simulink model "NeuroControlExamen"  (R2023b)
settings: Solver=VariableStepAuto  StartTime=0.0  StopTime=10.0  RelTol=1e-3
(part 2 of 3)

== matlab function NeuroControlExamen/Dinamica4 ==
  data: q input; qdd output; qd input; tau input
function qdd = fcn(q, qd, tau)

q1=q(1);
q2=q(2);
q3=q(3);
q1_d=qd(1);
q2_d=qd(2);
q3_d=qd(3);

m1 = 1;
m2 = 1;
m3 = 1;
l1 = 1;
l2 = 1;
l3 = 1;
lc1 = 0.5;
lc2 = 0.5;
lc3 = 0.5;
Ixx1 = 0.02;
Ixx2 = 0.02;
Ixx3 = 0.02;
Iyy1 = 0.02;
Iyy2 = 0.02;
Iyy3 = 0.02;
Izz1 = 0.02;
Izz2 = 0.02;
Izz3 = 0.02;

g = 9.81;

H = [Iyy1 + Ixx3*(cos(q2)*sin(q3) + cos(q3)*sin(q2))^2 + Iyy3*(cos(q2)*cos(q3) - sin(q2)*sin(q3))^2 + Iyy2*cos(q2)^2 + 2*m3*(l2*cos(q2)*sin(q1) + lc3*cos(q2)*cos(q3)*sin(q1) - lc3*sin(q1)*sin(q2)*sin(q3))^2 + Ixx2*sin(q2)^2 + lc2^2*m2*cos(q1)^2*cos(q2)^2 + lc2^2*m2*cos(q2)^2*sin(q1)^2, sin(q1)*(Ixx2*cos(q1)*cos(q2)*sin(q2) - Iyy2*cos(q1)*cos(q2)*sin(q2)) - cos(q1)*(Ixx2*cos(q2)*sin(q1)*sin(q2) - Iyy2*cos(q2)*sin(q1)*sin(q2)) + sin(q1)*(Ixx3*(cos(q1)*cos(q2)*cos(q3) - cos(q1)*sin(q2)*sin(q3))*(cos(q2)*sin(q3) + cos(q3)*sin(q2)) - Iyy3*(cos(q1)*cos(q2)*sin(q3) + cos(q1)*cos(q3)*sin(q2))*(cos(q2)*cos(q3) - sin(q2)*sin(q3))) + cos(q1)*(Ixx3*(sin(q1)*sin(q2)*sin(q3) - cos(q2)*cos(q3)*sin(q1))*(cos(q2)*sin(q3) + cos(q3)*sin(q2)) + Iyy3*(cos(q2)*sin(q1)*sin(q3) + cos(q3)*sin(q1)*sin(q2))*(cos(q2)*cos(q3) - sin(q2)*sin(q3))) + 2*m3*(l2*cos(q1)*sin(q2) + lc3*cos(q1)*cos(q2)*sin(q3) + lc3*cos(q1)*cos(q3)*sin(q2))*(l2*cos(q2)*sin(q1) + lc3*cos(q2)*cos(q3)*sin(q1) - lc3*sin(q1)*sin(q2)*sin(q3)), sin(q1)*(Ixx3*(cos(q1)*cos(q2)*cos(q3) - cos(q1)*sin(q2)*sin(q3))*(cos(q2)*sin(q3) + cos(q3)*sin(q2)) - Iyy3*(cos(q1)*cos(q2)*sin(q3) + cos(q1)*cos(q3)*sin(q2))*(cos(q2)*cos(q3) - sin(q2)*sin(q3))) + cos(q1)*(Ixx3*(sin(q1)*sin(q2)*sin(q3) - cos(q2)*cos(q3)*sin(q1))*(cos(q2)*sin(q3) + cos(q3)*sin(q2)) + Iyy3*(cos(q2)*sin(q1)*sin(q3) + cos(q3)*sin(q1)*sin(q2))*(cos(q2)*cos(q3) - sin(q2)*sin(q3))) + 2*m3*(lc3*cos(q1)*cos(q2)*sin(q3) + lc3*cos(q1)*cos(q3)*sin(q2))*(l2*cos(q2)*sin(q1) + lc3*cos(q2)*cos(q3)*sin(q1) - lc3*sin(q1)*sin(q2)*sin(q3));
     sin(q1)*(Ixx2*cos(q1)*cos(q2)*sin(q2) - Iyy2*cos(q1)*cos(q2)*sin(q2)) - cos(q1)*(Ixx2*cos(q2)*sin(q1)*sin(q2) - Iyy2*cos(q2)*sin(q1)*sin(q2)) + sin(q1)*(Ixx3*(cos(q1)*cos(q2)*cos(q3) - cos(q1)*sin(q2)*sin(q3))*(cos(q2)*sin(q3) + cos(q3)*sin(q2)) - Iyy3*(cos(q1)*cos(q2)*sin(q3) + cos(q1)*cos(q3)*sin(q2))*(cos(q2)*cos(q3) - sin(q2)*sin(q3))) + cos(q1)*(Ixx3*(sin(q1)*sin(q2)*sin(q3) - cos(q2)*cos(q3)*sin(q1))*(cos(q2)*sin(q3) + cos(q3)*sin(q2)) + Iyy3*(cos(q2)*sin(q1)*sin(q3) + cos(q3)*sin(q1)*sin(q2))*(cos(q2)*cos(q3) - sin(q2)*sin(q3))) + 2*m3*(l2*cos(q1)*sin(q2) + lc3*cos(q1)*cos(q2)*sin(q3) + lc3*cos(q1)*cos(q3)*sin(q2))*(l2*cos(q2)*sin(q1) + lc3*cos(q2)*cos(q3)*sin(q1) - lc3*sin(q1)*sin(q2)*sin(q3)), sin(q1)*(sin(q1)*(Ixx3*(cos(q1)*cos(q2)*cos(q3) - cos(q1)*sin(q2)*sin(q3))^2 + Iyy3*(cos(q1)*cos(q2)*sin(q3) + cos(q1)*cos(q3)*sin(q2))^2 + Izz3*sin(q1)^2) + cos(q1)*(Ixx3*(cos(q1)*cos(q2)*cos(q3) - cos(q1)*sin(q2)*sin(q3))*(sin(q1)*sin(q2)*sin(q3) - cos(q2)*cos(q3)*sin(q1)) - Iyy3*(cos(q1)*cos(q2)*sin(q3) + cos(q1)*cos(q3)*sin(q2))*(cos(q2)*sin(q1)*sin(q3) + cos(q3)*sin(q1)*sin(q2)) + Izz3*cos(q1)*sin(q1))) + cos(q1)*(cos(q1)*(Ixx3*(sin(q1)*sin(q2)*sin(q3) - cos(q2)*cos(q3)*sin(q1))^2 + Iyy3*(cos(q2)*sin(q1)*sin(q3) + cos(q3)*sin(q1)*sin(q2))^2 + Izz3*cos(q1)^2) + sin(q1)*(Ixx3*(cos(q1)*cos(q2)*cos(q3) - cos(q1)*sin(q2)*sin(q3))*(sin(q1)*sin(q2)*sin(q3) - cos(q2)*cos(q3)*sin(q1)) - Iyy3*(cos(q1)*cos(q2)*sin(q3) + cos(q1)*cos(q3)*sin(q2))*(cos(q2)*sin(q1)*sin(q3) + cos(q3)*sin(q1)*sin(q2)) + Izz3*cos(q1)*sin(q1))) - cos(q1)*(sin(q1)*(Ixx2*cos(q1)*cos(q2)^2*sin(q1) - Izz2*cos(q1)*sin(q1) + Iyy2*cos(q1)*sin(q1)*sin(q2)^2) - cos(q1)*(Izz2*cos(q1)^2 + Ixx2*cos(q2)^2*sin(q1)^2 + Iyy2*sin(q1)^2*sin(q2)^2)) - sin(q1)*(cos(q1)*(Ixx2*cos(q1)*cos(q2)^2*sin(q1) - Izz2*cos(q1)*sin(q1) + Iyy2*cos(q1)*sin(q1)*sin(q2)^2) - sin(q1)*(Ixx2*cos(q1)^2*cos(q2)^2 + Iyy2*cos(q1)^2*sin(q2)^2 + Izz2*sin(q1)^2)) + 2*m3*(l2*cos(q1)*sin(q2) + lc3*cos(q1)*cos(q2)*sin(q3) + lc3*cos(q1)*cos(q3)*sin(q2))^2 + m3*(cos(q2)*(l1 + l2) + lc3*cos(q2)*cos(q3) - lc3*sin(q2)*sin(q3))^2 + m2*cos(q2)^2*(l1 + lc2)^2 + lc2^2*m2*cos(q1)^2*sin(q2)^2 + lc2^2*m2*sin(q1)^2*sin(q2)^2, sin(q1)*(sin(q1)*(Ixx3*(cos(q1)*cos(q2)*cos(q3) - cos(q1)*sin(q2)*sin(q3))^2 + Iyy3*(cos(q1)*cos(q2)*sin(q3) + cos(q1)*cos(q3)*sin(q2))^2 + Izz3*sin(q1)^2) + cos(q1)*(Ixx3*(cos(q1)*cos(q2)*cos(q3) - cos(q1)*sin(q2)*sin(q3))*(sin(q1)*sin(q2)*sin(q3) - cos(q2)*cos(q3)*sin(q1)) - Iyy3*(cos(q1)*cos(q2)*sin(q3) + cos(q1)*cos(q3)*sin(q2))*(cos(q2)*sin(q1)*sin(q3) + cos(q3)*sin(q1)*sin(q2)) + Izz3*cos(q1)*sin(q1))) + cos(q1)*(cos(q1)*(Ixx3*(sin(q1)*sin(q2)*sin(q3) - cos(q2)*cos(q3)*sin(q1))^2 + Iyy3*(cos(q2)*sin(q1)*sin(q3) + cos(q3)*sin(q1)*sin(q2))^2 + Izz3*cos(q1)^2) + sin(q1)*(Ixx3*(cos(q1)*cos(q2)*cos(q3) - cos(q1)*sin(q2)*sin(q3))*(sin(q1)*sin(q2)*sin(q3) - cos(q2)*cos(q3)*sin(q1)) - Iyy3*(cos(q1)*cos(q2)*sin(q3) + cos(q1)*cos(q3)*sin(q2))*(cos(q2)*sin(q1)*sin(q3) + cos(q3)*sin(q1)*sin(q2)) + Izz3*cos(q1)*sin(q1))) + m3*(lc3*cos(q2)*cos(q3) - lc3*sin(q2)*sin(q3))*(cos(q2)*(l1 + l2) + lc3*cos(q2)*cos(q3) - lc3*sin(q2)*sin(q3)) + 2*m3*(lc3*cos(q1)*cos(q2)*sin(q3) + lc3*cos(q1)*cos(q3)*sin(q2))*(l2*cos(q1)*sin(q2) + lc3*cos(q1)*cos(q2)*sin(q3) + lc3*cos(q1)*cos(q3)*sin(q2));
     sin(q1)*(Ixx3*(cos(q1)*cos(q2)*cos(q3) - cos(q1)*sin(q2)*sin(q3))*(cos(q2)*sin(q3) + cos(q3)*sin(q2)) - Iyy3*(cos(q1)*cos(q2)*sin(q3) + cos(q1)*cos(q3)*sin(q2))*(cos(q2)*cos(q3) - sin(q2)*sin(q3))) + cos(q1)*(Ixx3*(sin(q1)*sin(q2)*sin(q3) - cos(q2)*cos(q3)*sin(q1))*(cos(q2)*sin(q3) + cos(q3)*sin(q2)) + Iyy3*(cos(q2)*sin(q1)*sin(q3) + cos(q3)*sin(q1)*sin(q2))*(cos(q2)*cos(q3) - sin(q2)*sin(q3))) + 2*m3*(lc3*cos(q1)*cos(q2)*sin(q3) + lc3*cos(q1)*cos(q3)*sin(q2))*(l2*cos(q2)*sin(q1) + lc3*cos(q2)*cos(q3)*sin(q1) - lc3*sin(q1)*sin(q2)*sin(q3)), sin(q1)*(sin(q1)*(Ixx3*(cos(q1)*cos(q2)*cos(q3) - cos(q1)*sin(q2)*sin(q3))^2 + Iyy3*(cos(q1)*cos(q2)*sin(q3) + cos(q1)*cos(q3)*sin(q2))^2 + Izz3*sin(q1)^2) + cos(q1)*(Ixx3*(cos(q1)*cos(q2)*cos(q3) - cos(q1)*sin(q2)*sin(q3))*(sin(q1)*sin(q2)*sin(q3) - cos(q2)*cos(q3)*sin(q1)) - Iyy3*(cos(q1)*cos(q2)*sin(q3) + cos(q1)*cos(q3)*sin(q2))*(cos(q2)*sin(q1)*sin(q3) + cos(q3)*sin(q1)*sin(q2)) + Izz3*cos(q1)*sin(q1))) + cos(q1)*(cos(q1)*(Ixx3*(sin(q1)*sin(q2)*sin(q3) - cos(q2)*cos(q3)*sin(q1))^2 + Iyy3*(cos(q2)*sin(q1)*sin(q3) + cos(q3)*sin(q1)*sin(q2))^2 + Izz3*cos(q1)^2) + sin(q1)*(Ixx3*(cos(q1)*cos(q2)*cos(q3) - cos(q1)*sin(q2)*sin(q3))*(sin(q1)*sin(q2)*sin(q3) - cos(q2)*cos(q3)*sin(q1)) - Iyy3*(cos(q1)*cos(q2)*sin(q3) + cos(q1)*cos(q3)*sin(q2))*(cos(q2)*sin(q1)*sin(q3) + cos(q3)*sin(q1)*sin(q2)) + Izz3*cos(q1)*sin(q1))) + m3*(lc3*cos(q2)*cos(q3) - lc3*sin(q2)*sin(q3))*(cos(q2)*(l1 + l2) + lc3*cos(q2)*cos(q3) - lc3*sin(q2)*sin(q3)) + 2*m3*(lc3*cos(q1)*cos(q2)*sin(q3) + lc3*cos(q1)*cos(q3)*sin(q2))*(l2*cos(q1)*sin(q2) + lc3*cos(q1)*cos(q2)*sin(q3) + lc3*cos(q1)*cos(q3)*sin(q2)), sin(q1)*(sin(q1)*(Ixx3*(cos(q1)*cos(q2)*cos(q3) - cos(q1)*sin(q2)*sin(q3))^2 + Iyy3*(cos(q1)*cos(q2)*sin(q3) + cos(q1)*cos(q3)*sin(q2))^2 + Izz3*sin(q1)^2) + cos(q1)*(Ixx3*(cos(q1)*cos(q2)*cos(q3) - cos(q1)*sin(q2)*sin(q3))*(sin(q1)*sin(q2)*sin(q3) - cos(q2)*cos(q3)*sin(q1)) - Iyy3*(cos(q1)*cos(q2)*sin(q3) + cos(q1)*cos(q3)*sin(q2))*(cos(q2)*sin(q1)*sin(q3) + cos(q3)*sin(q1)*sin(q2)) + Izz3*cos(q1)*sin(q1))) + 2*m3*(lc3*cos(q1)*cos(q2)*sin(q3) + lc3*cos(q1)*cos(q3)*sin(q2))^2 + cos(q1)*(cos(q1)*(Ixx3*(sin(q1)*sin(q2)*sin(q3) - cos(q2)*cos(q3)*sin(q1))^2 + Iyy3*(cos(q2)*sin(q1)*sin(q3) + cos(q3)*sin(q1)*sin(q2))^2 + Izz3*cos(q1)^2) + sin(q1)*(Ixx3*(cos(q1)*cos(q2)*cos(q3) - cos(q1)*sin(q2)*sin(q3))*(sin(q1)*sin(q2)*sin(q3) - cos(q2)*cos(q3)*sin(q1)) - Iyy3*(cos(q1)*cos(q2)*sin(q3) + cos(q1)*cos(q3)*sin(q2))*(cos(q2)*sin(q1)*sin(q3) + cos(q3)*sin(q1)*sin(q2)) + Izz3*cos(q1)*sin(q1))) + m3*(lc3*cos(q2)*cos(q3) - lc3*sin(q2)*sin(q3))^2];
 
g_q = [g*m2*(lc2*cos(q1 + q2) + l1*cos(q1)) + g*lc1*m1*cos(q1);
       g*lc2*m2*cos(q1 + q2);
       0];

C = [2*m3*q1_d*(l2*cos(q1)*cos(q2) + lc3*cos(q1)*cos(q2)*cos(q3) - lc3*cos(q1)*sin(q2)*sin(q3))*(l2*cos(q2)*sin(q1) + lc3*cos(q2)*cos(q3)*sin(q1) - lc3*sin(q1)*sin(q2)*sin(q3)) - q2_d*(2*m3*(l2*cos(q2)*sin(q1) + lc3*cos(q2)*cos(q3)*sin(q1) - lc3*sin(q1)*sin(q2)*sin(q3))*(l2*sin(q1)*sin(q2) + lc3*cos(q2)*sin(q1)*sin(q3) + lc3*cos(q3)*sin(q1)*sin(q2)) - Ixx2*cos(q2)*sin(q2) + Iyy2*cos(q2)*sin(q2) - Ixx3*(cos(q2)*sin(q3) + cos(q3)*sin(q2))*(cos(q2)*cos(q3) - sin(q2)*sin(q3)) + Iyy3*(cos(q2)*sin(q3) + cos(q3)*sin(q2))*(cos(q2)*cos(q3) - sin(q2)*sin(q3)) + lc2^2*m2*cos(q1)^2*cos(q2)*sin(q2) + lc2^2*m2*cos(q2)*sin(q1)^2*sin(q2)) - q3_d*(2*m3*(lc3*cos(q2)*sin(q1)*sin(q3) + lc3*cos(q3)*sin(q1)*sin(q2))*(l2*cos(q2)*sin(q1) + lc3*cos(q2)*cos(q3)*sin(q1) - lc3*sin(q1)*sin(q2)*sin(q3)) - Ixx3*(cos(q2)*sin(q3) + cos(q3)*sin(q2))*(cos(q2)*cos(q3) - sin(q2)*sin(q3)) + Iyy3*(cos(q2)*sin(q3) + cos(q3)*sin(q2))*(cos(q2)*cos(q3) - sin(q2)*sin(q3))), q2_d*((sin(q1)*(cos(q1)*(Ixx3*(sin(q1)*sin(q2)*sin(q3) - cos(q2)*cos(q3)*sin(q1))^2 + Iyy3*(cos(q2)*sin(q1)*sin(q3) + cos(q3)*sin(q1)*sin(q2))^2 + Izz3*cos(q1)^2) + sin(q1)*(Ixx3*(cos(q1)*cos(q2)*cos(q3) - cos(q1)*sin(q2)*sin(q3))*(sin(q1)*sin(q2)*sin(q3) - cos(q2)*cos(q3)*sin(q1)) - Iyy3*(cos(q1)*cos(q2)*sin(q3) + cos(q1)*cos(q3)*sin(q2))*(cos(q2)*sin(q1)*sin(q3) + cos(q3)*sin(q1)*sin(q2)) + Izz3*cos(q1)*sin(q1))))/2 - (sin(q1)*(cos(q1)*(Ixx3*(cos(q1)*cos(q2)*cos(q3) - cos(q1)*sin(q2)*sin(q3))^2 + Iyy3*(cos(q1)*cos(q2)*sin(q3) + cos(q1)*cos(q3)*sin(q2))^2 + Izz3*sin(q1)^2) - sin(q1)*(Ixx3*(cos(q1)*cos(q2)*cos(q3) - cos(q1)*sin(q2)*sin(q3))*(sin(q1)*sin(q2)*sin(q3) - cos(q2)*cos(q3)*sin(q1)) - Iyy3*(cos(q1)*cos(q2)*sin(q3) + cos(q1)*cos(q3)*sin(q2))*(cos(q2)*sin(q1)*sin(q3) + cos(q3)*sin(q1)*sin(q2)) + Izz3*cos(q1)*sin(q1)) + sin(q1)*(2*Ixx3*(cos(q1)*cos(q2)*cos(q3) - cos(q1)*sin(q2)*sin(q3))*(sin(q1)*sin(q2)*sin(q3) - cos(q2)*cos(q3)*sin(q1)) - 2*Iyy3*(cos(q1)*cos(q2)*sin(q3) + cos(q1)*cos(q3)*sin(q2))*(cos(q2)*sin(q1)*sin(q3) + cos(q3)*sin(q1)*sin(q2)) + 2*Izz3*cos(q1)*sin(q1)) - cos(q1)*(Ixx3*(cos(q1)*cos(q2)*cos(q3) - cos(q1)*sin(q2)*sin(q3))^2 + Iyy3*(cos(q1)*cos(q2)*sin(q3) + cos(q1)*cos(q3)*sin(q2))^2 - Ixx3*(sin(q1)*sin(q2)*sin(q3) - cos(q2)*cos(q3)*sin(q1))^2 - Iyy3*(cos(q2)*sin(q1)*sin(q3) + cos(q3)*sin(q1)*sin(q2))^2 - Izz3*cos(q1)^2 + Izz3*sin(q1)^2)))/2 - (cos(q1)*(sin(q1)*(Ixx3*(cos(q1)*cos(q2)*cos(q3) - cos(q1)*sin(q2)*sin(q3))^2 + Iyy3*(cos(q1)*cos(q2)*sin(q3) + cos(q1)*cos(q3)*sin(q2))^2 + Izz3*sin(q1)^2) + cos(q1)*(Ixx3*(cos(q1)*cos(q2)*cos(q3) - cos(q1)*sin(q2)*sin(q3))*(sin(q1)*sin(q2)*sin(q3) - cos(q2)*cos(q3)*sin(q1)) - Iyy3*(cos(q1)*cos(q2)*sin(q3) + cos(q1)*cos(q3)*sin(q2))*(cos(q2)*sin(q1)*sin(q3) + cos(q3)*sin(q1)*sin(q2)) + Izz3*cos(q1)*sin(q1))))/2 + (cos(q1)*(sin(q1)*(Ixx3*(sin(q1)*sin(q2)*sin(q3) - cos(q2)*cos(q3)*sin(q1))^2 + Iyy3*(cos(q2)*sin(q1)*sin(q3) + cos(q3)*sin(q1)*sin(q2))^2 + Izz3*cos(q1)^2) - cos(q1)*(Ixx3*(cos(q1)*cos(q2)*cos(q3) - cos(q1)*sin(q2)*sin(q3))*(sin(q1)*sin(q2)*sin(q3) - cos(q2)*cos(q3)*sin(q1)) - Iyy3*(cos(q1)*cos(q2)*sin(q3) + cos(q1)*cos(q3)*sin(q2))*(cos(q2)*sin(q1)*sin(q3) + cos(q3)*sin(q1)*sin(q2)) + Izz3*cos(q1)*sin(q1)) + cos(q1)*(2*Ixx3*(cos(q1)*cos(q2)*cos(q3) - cos(q1)*sin(q2)*sin(q3))*(sin(q1)*sin(q2)*sin(q3) - cos(q2)*cos(q3)*sin(q1)) - 2*Iyy3*(cos(q1)*cos(q2)*sin(q3) + cos(q1)*cos(q3)*sin(q2))*(cos(q2)*sin(q1)*sin(q3) + cos(q3)*sin(q1)*sin(q2)) + 2*Izz3*cos(q1)*sin(q1)) + sin(q1)*(Ixx3*(cos(q1)*cos(q2)*cos(q3) - cos(q1)*sin(q2)*sin(q3))^2 + Iyy3*(cos(q1)*cos(q2)*sin(q3) + cos(q1)*cos(q3)*sin(q2))^2 - Ixx3*(sin(q1)*sin(q2)*sin(q3) - cos(q2)*cos(q3)*sin(q1))^2 - Iyy3*(cos(q2)*sin(q1)*sin(q3) + cos(q3)*sin(q1)*sin(q2))^2 - Izz3*cos(q1)^2 + Izz3*sin(q1)^2)))/2 - sin(q1)*(Ixx3*(cos(q1)*cos(q2)*sin(q3) + cos(q1)*cos(q3)*sin(q2))*(cos(q2)*sin(q3) + cos(q3)*sin(q2)) - Ixx3*(cos(q1)*cos(q2)*cos(q3) - cos(q1)*sin(q2)*sin(q3))*(cos(q2)*cos(q3) - sin(q2)*sin(q3)) - Iyy3*(cos(q1)*cos(q2)*sin(q3) + cos(q1)*cos(q3)*sin(q2))*(cos(q2)*sin(q3) + cos(q3)*sin(q2)) + Iyy3*(cos(q1)*cos(q2)*cos(q3) - cos(q1)*sin(q2)*sin(q3))*(cos(q2)*cos(q3) - sin(q2)*sin(q3))) + (cos(q1)*(cos(q1)*(Ixx2*cos(q1)*cos(q2)^2*sin(q1) - Izz2*cos(q1)*sin(q1) + Iyy2*cos(q1)*sin(q1)*sin(q2)^2) - sin(q1)*(Ixx2*cos(q1)^2*cos(q2)^2 + Iyy2*cos(q1)^2*sin(q2)^2 + Izz2*sin(q1)^2)))/2 + sin(q1)*(Ixx2*cos(q1)*cos(q2)^2 - Iyy2*cos(q1)*cos(q2)^2 - Ixx2*cos(q1)*sin(q2)^2 + Iyy2*cos(q1)*sin(q2)^2) - (sin(q1)*(sin(q1)*(Ixx2*cos(q1)*cos(q2)^2*sin(q1) - Izz2*cos(q1)*sin(q1) + Iyy2*cos(q1)*sin(q1)*sin(q2)^2) - cos(q1)*(Izz2*cos(q1)^2 + Ixx2*cos(q2)^2*sin(q1)^2 + Iyy2*sin(q1)^2*sin(q2)^2)))/2 - (sin(q1)*(sin(q1)*(Ixx2*cos(q1)*cos(q2)^2*sin(q1) - Izz2*cos(q1)*sin(q1) + Iyy2*cos(q1)*sin(q1)*sin(q2)^2) - sin(q1)*(2*Ixx2*cos(q1)*cos(q2)^2*sin(q1) - 2*Izz2*cos(q1)*sin(q1) + 2*Iyy2*cos(q1)*sin(q1)*sin(q2)^2) + cos(q1)*(Ixx2*cos(q1)^2*cos(q2)^2 + Iyy2*cos(q1)^2*sin(q2)^2 + Izz2*sin(q1)^2) + cos(q1)*(- Ixx2*cos(q1)^2*cos(q2)^2 - Iyy2*cos(q1)^2*sin(q2)^2 + Izz2*cos(q1)^2 + Ixx2*cos(q2)^2*sin(q1)^2 + Iyy2*sin(q1)^2*sin(q2)^2 - Izz2*sin(q1)^2)))/2 + (cos(q1)*(cos(q1)*(Ixx2*cos(q1)*cos(q2)^2*sin(q1) - Izz2*cos(q1)*sin(q1) + Iyy2*cos(q1)*sin(q1)*sin(q2)^2) - cos(q1)*(2*Ixx2*cos(q1)*cos(q2)^2*sin(q1) - 2*Izz2*cos(q1)*sin(q1) + 2*Iyy2*cos(q1)*sin(q1)*sin(q2)^2) + sin(q1)*(Izz2*cos(q1)^2 + Ixx2*cos(q2)^2*sin(q1)^2 + Iyy2*sin(q1)^2*sin(q2)^2) - sin(q1)*(- Ixx2*cos(q1)^2*cos(q2)^2 - Iyy2*cos(q1)^2*sin(q2)^2 + Izz2*cos(q1)^2 + Ixx2*cos(q2)^2*sin(q1)^2 + Iyy2*sin(q1)^2*sin(q2)^2 - Izz2*sin(q1)^2)))/2 - cos(q1)*(Ixx2*cos(q2)^2*sin(q1) - Iyy2*cos(q2)^2*sin(q1) - Ixx2*sin(q1)*sin(q2)^2 + Iyy2*sin(q1)*sin(q2)^2) + cos(q1)*(Ixx3*(cos(q2)*sin(q1)*sin(q3) + cos(q3)*sin(q1)*sin(q2))*(cos(q2)*sin(q3) + cos(q3)*sin(q2)) + Ixx3*(sin(q1)*sin(q2)*sin(q3) - cos(q2)*cos(q3)*sin(q1))*(cos(q2)*cos(q3) - sin(q2)*sin(q3)) - Iyy3*(cos(q2)*sin(q1)*sin(q3) + cos(q3)*sin(q1)*sin(q2))*(cos(q2)*sin(q3) + cos(q3)*sin(q2)) - Iyy3*(sin(q1)*sin(q2)*sin(q3) - cos(q2)*cos(q3)*sin(q1))*(cos(q2)*cos(q3) - sin(q2)*sin(q3))) + 2*m3*(l2*cos(q1)*cos(q2) + lc3*cos(q1)*cos(q2)*cos(q3) - lc3*cos(q1)*sin(q2)*sin(q3))*(l2*cos(q2)*sin(q1) + lc3*cos(q2)*cos(q3)*sin(q1) - lc3*sin(q1)*sin(q2)*sin(q3))) - q1_d*(2*m3*(l2*cos(q2)*sin(q1) + lc3*cos(q2)*cos(q3)*sin(q1) - lc3*sin(q1)*sin(q2)*sin(q3))*(l2*sin(q1)*sin(q2) + lc3*cos(q2)*sin(q1)*sin(q3) + lc3*cos(q3)*sin(q1)*sin(q2)) - Ixx2*cos(q2)*sin(q2) + Iyy2*cos(q2)*sin(q2) - Ixx3*(cos(q2)*sin(q3) + cos(q3)*sin(q2))*(cos(q2)*cos(q3) - sin(q2)*sin(q3)) + Iyy3*(cos(q2)*sin(q3) + cos(q3)*sin(q2))*(cos(q2)*cos(q3) - sin(q2)*sin(q3)) + lc2^2*m2*cos(q1)^2*cos(q2)*sin(q2) + lc2^2*m2*cos(q2)*sin(q1)^2*sin(q2)) + q3_d*((sin(q1)*(cos(q1)*(Ixx3*(sin(q1)*sin(q2)*sin(q3) - cos(q2)*cos(q3)*sin(q1))^2 + Iyy3*(cos(q2)*sin(q1)*sin(q3) + cos(q3)*sin(q1)*sin(q2))^2 + Izz3*cos(q1)^2) + sin(q1)*(Ixx3*(cos(q1)*cos(q2)*cos(q3) - cos(q1)*sin(q2)*sin(q3))*(sin(q1)*sin(q2)*sin(q3) - cos(q2)*cos(q3)*sin(q1)) - Iyy3*(cos(q1)*cos(q2)*sin(q3) + cos(q1)*cos(q3)*sin(q2))*(cos(q2)*sin(q1)*sin(q3) + cos(q3)*sin(q1)*sin(q2)) + Izz3*cos(q1)*sin(q1))))/2 - (sin(q1)*(cos(q1)*(Ixx3*(cos(q1)*cos(q2)*cos(q3) - cos(q1)*sin(q2)*sin(q3))^2 + Iyy3*(cos(q1)*cos(q2)*sin(q3) + cos(q1)*cos(q3)*sin(q2))^2 + Izz3*sin(q1)^2) - sin(q1)*(Ixx3*(cos(q1)*cos(q2)*cos(q3) - cos(q1)*sin(q2)*sin(q3))*(sin(q1)*sin(q2)*sin(q3) - cos(q2)*cos(q3)*sin(q1)) - Iyy3*(cos(q1)*cos(q2)*sin(q3) + cos(q1)*cos(q3)*sin(q2))*(cos(q2)*sin(q1)*sin(q3) + cos(q3)*sin(q1)*sin(q2)) + Izz3*cos(q1)*sin(q1)) + sin(q1)*(2*Ixx3*(cos(q1)*cos(q2)*cos(q3) - cos(q1)*sin(q2)*sin(q3))*(sin(q1)*sin(q2)*sin(q3) - cos(q2)*cos(q3)*sin(q1)) - 2*Iyy3*(cos(q1)*cos(q2)*sin(q3) + cos(q1)*cos(q3)*sin(q2))*(cos(q2)*sin(q1)*sin(q3) + cos(q3)*sin(q1)*sin(q2)) + 2*Izz3*cos(q1)*sin(q1)) - cos(q1)*(Ixx3*(cos(q1)*cos(q2)*cos(q3) - cos(q1)*sin(q2)*sin(q3))^2 + Iyy3*(cos(q1)*cos(q2)*sin(q3) + cos(q1)*cos(q3)*sin(q2))^2 - Ixx3*(sin(q1)*sin(q2)*sin(q3) - cos(q2)*cos(q3)*sin(q1))^2 - Iyy3*(cos(q2)*sin(q1)*sin(q3) + cos(q3)*sin(q1)*sin(q2))^2 - Izz3*cos(q1)^2 + Izz3*sin(q1)^2)))/2 - (cos(q1)*(sin(q1)*(Ixx3*(cos(q1)*cos(q2)*cos(q3) - cos(q1)*sin(q2)*sin(q3))^2 + Iyy3*(cos(q1)*cos(q2)*sin(q3) + cos(q1)*cos(q3)*sin(q2))^2 + Izz3*sin(q1)^2) + cos(q1)*(Ixx3*(cos(q1)*cos(q2)*cos(q3) - cos(q1)*sin(q2)*sin(q3))*(sin(q1)*sin(q2)*sin(q3) - cos(q2)*cos(q3)*sin(q1)) - Iyy3*(cos(q1)*cos(q2)*sin(q3) + cos(q1)*cos(q3)*sin(q2))*(cos(q2)*sin(q1)*sin(q3) + cos(q3)*sin(q1)*sin(q2)) + Izz3*cos(q1)*sin(q1))))/2 + (cos(q1)*(sin(q1)*(Ixx3*(sin(q1)*sin(q2)*sin(q3) - cos(q2)*cos(q3)*sin(q1))^2 + Iyy3*(cos(q2)*sin(q1)*sin(q3) + cos(q3)*sin(q1)*sin(q2))^2 + Izz3*cos(q1)^2) - cos(q1)*(Ixx3*(cos(q1)*cos(q2)*cos(q3) - cos(q1)*sin(q2)*sin(q3))*(sin(q1)*sin(q2)*sin(q3) - cos(q2)*cos(q3)*sin(q1)) - Iyy3*(cos(q1)*cos(q2)*sin(q3) + cos(q1)*cos(q3)*sin(q2))*(cos(q2)*sin(q1)*sin(q3) + cos(q3)*sin(q1)*sin(q2)) + Izz3*cos(q1)*sin(q1)) + cos(q1)*(2*Ixx3*(cos(q1)*cos(q2)*cos(q3) - cos(q1)*sin(q2)*sin(q3))*(sin(q1)*sin(q2)*sin(q3) - cos(q2)*cos(q3)*sin(q1)) - 2*Iyy3*(cos(q1)*cos(q2)*sin(q3) + cos(q1)*cos(q3)*sin(q2))*(cos(q2)*sin(q1)*sin(q3) + cos(q3)*sin(q1)*sin(q2)) + 2*Izz3*cos(q1)*sin(q1)) + sin(q1)*(Ixx3*(cos(q1)*cos(q2)*cos(q3) - cos(q1)*sin(q2)*sin(q3))^2 + Iyy3*(cos(q1)*cos(q2)*sin(q3) + cos(q1)*cos(q3)*sin(q2))^2 - Ixx3*(sin(q1)*sin(q2)*sin(q3) - cos(q2)*cos(q3)*sin(q1))^2 - Iyy3*(cos(q2)*sin(q1)*sin(q3) + cos(q3)*sin(q1)*sin(q2))^2 - Izz3*cos(q1)^2 + Izz3*sin(q1)^2)))/2 - sin(q1)*(Ixx3*(cos(q1)*cos(q2)*sin(q3) + cos(q1)*cos(q3)*sin(q2))*(cos(q2)*sin(q3) + cos(q3)*sin(q2)) - Ixx3*(cos(q1)*cos(q2)*cos(q3) - cos(q1)*sin(q2)*sin(q3))*(cos(q2)*cos(q3) - sin(q2)*sin(q3)) - Iyy3*(cos(q1)*cos(q2)*sin(q3) + cos(q1)*cos(q3)*sin(q2))*(cos(q2)*sin(q3) + cos(q3)*sin(q2)) + Iyy3*(cos(q1)*cos(q2)*cos(q3) - cos(q1)*sin(q2)*sin(q3))*(cos(q2)*cos(q3) - sin(q2)*sin(q3))) + cos(q1)*(Ixx3*(cos(q2)*sin(q1)*sin(q3) + cos(q3)*sin(q1)*sin(q2))*(cos(q2)*sin(q3) + cos(q3)*sin(q2)) + Ixx3*(sin(q1)*sin(q2)*sin(q3) - cos(q2)*cos(q3)*sin(q1))*(cos(q2)*cos(q3) - sin(q2)*sin(q3)) - Iyy3*(cos(q2)*sin(q1)*sin(q3) + cos(q3)*sin(q1)*sin(q2))*(cos(q2)*sin(q3) + cos(q3)*sin(q2)) - Iyy3*(sin(q1)*sin(q2)*sin(q3) - cos(q2)*cos(q3)*sin(q1))*(cos(q2)*cos(q3) - sin(q2)*sin(q3))) + 2*m3*(lc3*cos(q1)*cos(q2)*cos(q3) - lc3*cos(q1)*sin(q2)*sin(q3))*(l2*cos(q2)*sin(q1) + lc3*cos(q2)*cos(q3)*sin(q1) - lc3*sin(q1)*sin(q2)*sin(q3))), q3_d*((cos(q1)*(sin(q1)*(Ixx3*(cos(q1)*cos(q2)*cos(q3) - cos(q1)*sin(q2)*sin(q3))^2 + Iyy3*(cos(q1)*cos(q2)*sin(q3) + cos(q1)*cos(q3)*sin(q2))^2 + Izz3*sin(q1)^2) + cos(q1)*(Ixx3*(cos(q1)*cos(q2)*cos(q3) - cos(q1)*sin(q2)*sin(q3))*(sin(q1)*sin(q2)*sin(q3) - cos(q2)*cos(q3)*sin(q1)) - Iyy3*(cos(q1)*cos(q2)*sin(q3) + cos(q1)*cos(q3)*sin(q2))*(cos(q2)*sin(q1)*sin(q3) + cos(q3)*sin(q1)*sin(q2)) + Izz3*cos(q1)*sin(q1))))/2 + (sin(q1)*(cos(q1)*(Ixx3*(cos(q1)*cos(q2)*cos(q3) - cos(q1)*sin(q2)*sin(q3))^2 + Iyy3*(cos(q1)*cos(q2)*sin(q3) + cos(q1)*cos(q3)*sin(q2))^2 + Izz3*sin(q1)^2) - sin(q1)*(Ixx3*(cos(q1)*cos(q2)*cos(q3) - cos(q1)*sin(q2)*sin(q3))*(sin(q1)*sin(q2)*sin(q3) - cos(q2)*cos(q3)*sin(q1)) - Iyy3*(cos(q1)*cos(q2)*sin(q3) + cos(q1)*cos(q3)*sin(q2))*(cos(q2)*sin(q1)*sin(q3) + cos(q3)*sin(q1)*sin(q2)) + Izz3*cos(q1)*sin(q1)) + sin(q1)*(2*Ixx3*(cos(q1)*cos(q2)*cos(q3) - cos(q1)*sin(q2)*sin(q3))*(sin(q1)*sin(q2)*sin(q3) - cos(q2)*cos(q3)*sin(q1)) - 2*Iyy3*(cos(q1)*cos(q2)*sin(q3) + cos(q1)*cos(q3)*sin(q2))*(cos(q2)*sin(q1)*sin(q3) + cos(q3)*sin(q1)*sin(q2)) + 2*Izz3*cos(q1)*sin(q1)) - cos(q1)*(Ixx3*(cos(q1)*cos(q2)*cos(q3) - cos(q1)*sin(q2)*sin(q3))^2 + Iyy3*(cos(q1)*cos(q2)*sin(q3) + cos(q1)*cos(q3)*sin(q2))^2 - Ixx3*(sin(q1)*sin(q2)*sin(q3) - cos(q2)*cos(q3)*sin(q1))^2 - Iyy3*(cos(q2)*sin(q1)*sin(q3) + cos(q3)*sin(q1)*sin(q2))^2 - Izz3*cos(q1)^2 + Izz3*sin(q1)^2)))/2 - (sin(q1)*(cos(q1)*(Ixx3*(sin(q1)*sin(q2)*sin(q3) - cos(q2)*cos(q3)*sin(q1))^2 + Iyy3*(cos(q2)*sin(q1)*sin(q3) + cos(q3)*sin(q1)*sin(q2))^2 + Izz3*cos(q1)^2) + sin(q1)*(Ixx3*(cos(q1)*cos(q2)*cos(q3) - cos(q1)*sin(q2)*sin(q3))*(sin(q1)*sin(q2)*sin(q3) - cos(q2)*cos(q3)*sin(q1)) - Iyy3*(cos(q1)*cos(q2)*sin(q3) + cos(q1)*cos(q3)*sin(q2))*(cos(q2)*sin(q1)*sin(q3) + cos(q3)*sin(q1)*sin(q2)) + Izz3*cos(q1)*sin(q1))))/2 - (cos(q1)*(sin(q1)*(Ixx3*(sin(q1)*sin(q2)*sin(q3) - cos(q2)*cos(q3)*sin(q1))^2 + Iyy3*(cos(q2)*sin(q1)*sin(q3) + cos(q3)*sin(q1)*sin(q2))^2 + Izz3*cos(q1)^2) - cos(q1)*(Ixx3*(cos(q1)*cos(q2)*cos(q3) - cos(q1)*sin(q2)*sin(q3))*(sin(q1)*sin(q2)*sin(q3) - cos(q2)*cos(q3)*sin(q1)) - Iyy3*(cos(q1)*cos(q2)*sin(q3) + cos(q1)*cos(q3)*sin(q2))*(cos(q2)*sin(q1)*sin(q3) + cos(q3)*sin(q1)*sin(q2)) + Izz3*cos(q1)*sin(q1)) + cos(q1)*(2*Ixx3*(cos(q1)*cos(q2)*cos(q3) - cos(q1)*sin(q2)*sin(q3))*(sin(q1)*sin(q2)*sin(q3) - cos(q2)*cos(q3)*sin(q1)) - 2*Iyy3*(cos(q1)*cos(q2)*sin(q3) + cos(q1)*cos(q3)*sin(q2))*(cos(q2)*sin(q1)*sin(q3) + cos(q3)*sin(q1)*sin(q2)) + 2*Izz3*cos(q1)*sin(q1)) + sin(q1)*(Ixx3*(cos(q1)*cos(q2)*cos(q3) - cos(q1)*sin(q2)*sin(q3))^2 + Iyy3*(cos(q1)*cos(q2)*sin(q3) + cos(q1)*cos(q3)*sin(q2))^2 - Ixx3*(sin(q1)*sin(q2)*sin(q3) - cos(q2)*cos(q3)*sin(q1))^2 - Iyy3*(cos(q2)*sin(q1)*sin(q3) + cos(q3)*sin(q1)*sin(q2))^2 - Izz3*cos(q1)^2 + Izz3*sin(q1)^2)))/2 - sin(q1)*(Ixx3*(cos(q1)*cos(q2)*sin(q3) + cos(q1)*cos(q3)*sin(q2))*(cos(q2)*sin(q3) + cos(q3)*sin(q2)) - Ixx3*(cos(q1)*cos(q2)*cos(q3) - cos(q1)*sin(q2)*sin(q3))*(cos(q2)*cos(q3) - sin(q2)*sin(q3)) - Iyy3*(cos(q1)*cos(q2)*sin(q3) + cos(q1)*cos(q3)*sin(q2))*(cos(q2)*sin(q3) + cos(q3)*sin(q2)) + Iyy3*(cos(q1)*cos(q2)*cos(q3) - cos(q1)*sin(q2)*sin(q3))*(cos(q2)*cos(q3) - sin(q2)*sin(q3))) + cos(q1)*(Ixx3*(cos(q2)*sin(q1)*sin(q3) + cos(q3)*sin(q1)*sin(q2))*(cos(q2)*sin(q3) + cos(q3)*sin(q2)) + Ixx3*(sin(q1)*sin(q2)*sin(q3) - cos(q2)*cos(q3)*sin(q1))*(cos(q2)*cos(q3) - sin(q2)*sin(q3)) - Iyy3*(cos(q2)*sin(q1)*sin(q3) + cos(q3)*sin(q1)*sin(q2))*(cos(q2)*sin(q3) + cos(q3)*sin(q2)) - Iyy3*(sin(q1)*sin(q2)*sin(q3) - cos(q2)*cos(q3)*sin(q1))*(cos(q2)*cos(q3) - sin(q2)*sin(q3))) - 4*m3*(lc3*cos(q1)*cos(q2)*sin(q3) + lc3*cos(q1)*cos(q3)*sin(q2))*(lc3*cos(q2)*sin(q1)*sin(q3) + lc3*cos(q3)*sin(q1)*sin(q2)) + 2*m3*(lc3*cos(q1)*cos(q2)*cos(q3) - lc3*cos(q1)*sin(q2)*sin(q3))*(l2*cos(q2)*sin(q1) + lc3*cos(q2)*cos(q3)*sin(q1) - lc3*sin(q1)*sin(q2)*sin(q3))) - q2_d*((sin(q1)*(cos(q1)*(Ixx3*(sin(q1)*sin(q2)*sin(q3) - cos(q2)*cos(q3)*sin(q1))^2 + Iyy3*(cos(q2)*sin(q1)*sin(q3) + cos(q3)*sin(q1)*sin(q2))^2 + Izz3*cos(q1)^2) + sin(q1)*(Ixx3*(cos(q1)*cos(q2)*cos(q3) - cos(q1)*sin(q2)*sin(q3))*(sin(q1)*sin(q2)*sin(q3) - cos(q2)*cos(q3)*sin(q1)) - Iyy3*(cos(q1)*cos(q2)*sin(q3) + cos(q1)*cos(q3)*sin(q2))*(cos(q2)*sin(q1)*sin(q3) + cos(q3)*sin(q1)*sin(q2)) + Izz3*cos(q1)*sin(q1))))/2 - (sin(q1)*(cos(q1)*(Ixx3*(cos(q1)*cos(q2)*cos(q3) - cos(q1)*sin(q2)*sin(q3))^2 + Iyy3*(cos(q1)*cos(q2)*sin(q3) + cos(q1)*cos(q3)*sin(q2))^2 + Izz3*sin(q1)^2) - sin(q1)*(Ixx3*(cos(q1)*cos(q2)*cos(q3) - cos(q1)*sin(q2)*sin(q3))*(sin(q1)*sin(q2)*sin(q3) - cos(q2)*cos(q3)*sin(q1)) - Iyy3*(cos(q1)*cos(q2)*sin(q3) + cos(q1)*cos(q3)*sin(q2))*(cos(q2)*sin(q1)*sin(q3) + cos(q3)*sin(q1)*sin(q2)) + Izz3*cos(q1)*sin(q1)) + sin(q1)*(2*Ixx3*(cos(q1)*cos(q2)*cos(q3) - cos(q1)*sin(q2)*sin(q3))*(sin(q1)*sin(q2)*sin(q3) - cos(q2)*cos(q3)*sin(q1)) - 2*Iyy3*(cos(q1)*cos(q2)*sin(q3) + cos(q1)*cos(q3)*sin(q2))*(cos(q2)*sin(q1)*sin(q3) + cos(q3)*sin(q1)*sin(q2)) + 2*Izz3*cos(q1)*sin(q1)) - cos(q1)*(Ixx3*(cos(q1)*cos(q2)*cos(q3) - cos(q1)*sin(q2)*sin(q3))^2 + Iyy3*(cos(q1)*cos(q2)*sin(q3) + cos(q1)*cos(q3)*sin(q2))^2 - Ixx3*(sin(q1)*sin(q2)*sin(q3) - cos(q2)*cos(q3)*sin(q1))^2 - Iyy3*(cos(q2)*sin(q1)*sin(q3) + cos(q3)*sin(q1)*sin(q2))^2 - Izz3*cos(q1)^2 + Izz3*sin(q1)^2)))/2 - (cos(q1)*(sin(q1)*(Ixx3*(cos(q1)*cos(q2)*cos(q3) - cos(q1)*sin(q2)*sin(q3))^2 + Iyy3*(cos(q1)*cos(q2)*sin(q3) + cos(q1)*cos(q3)*sin(q2))^2 + Izz3*sin(q1)^2) + cos(q1)*(Ixx3*(cos(q1)*cos(q2)*cos(q3) - cos(q1)*sin(q2)*sin(q3))*(sin(q1)*sin(q2)*sin(q3) - cos(q2)*cos(q3)*sin(q1)) - Iyy3*(cos(q1)*cos(q2)*sin(q3) + cos(q1)*cos(q3)*sin(q2))*(cos(q2)*sin(q1)*sin(q3) + cos(q3)*sin(q1)*sin(q2)) + Izz3*cos(q1)*sin(q1))))/2 + (cos(q1)*(sin(q1)*(Ixx3*(sin(q1)*sin(q2)*sin(q3) - cos(q2)*cos(q3)*sin(q1))^2 + Iyy3*(cos(q2)*sin(q1)*sin(q3) + cos(q3)*sin(q1)*sin(q2))^2 + Izz3*cos(q1)^2) - cos(q1)*(Ixx3*(cos(q1)*cos(q2)*cos(q3) - cos(q1)*sin(q2)*sin(q3))*(sin(q1)*sin(q2)*sin(q3) - cos(q2)*cos(q3)*sin(q1)) - Iyy3*(cos(q1)*cos(q2)*sin(q3) + cos(q1)*cos(q3)*sin(q2))*(cos(q2)*sin(q1)*sin(q3) + cos(q3)*sin(q1)*sin(q2)) + Izz3*cos(q1)*sin(q1)) + cos(q1)*(2*Ixx3*(cos(q1)*cos(q2)*cos(q3) - cos(q1)*sin(q2)*sin(q3))*(sin(q1)*sin(q2)*sin(q3) - cos(q2)*cos(q3)*sin(q1)) - 2*Iyy3*(cos(q1)*cos(q2)*sin(q3) + cos(q1)*cos(q3)*sin(q2))*(cos(q2)*sin(q1)*sin(q3) + cos(q3)*sin(q1)*sin(q2)) + 2*Izz3*cos(q1)*sin(q1)) + sin(q1)*(Ixx3*(cos(q1)*cos(q2)*cos(q3) - cos(q1)*sin(q2)*sin(q3))^2 + Iyy3*(cos(q1)*cos(q2)*sin(q3) + cos(q1)*cos(q3)*sin(q2))^2 - Ixx3*(sin(q1)*sin(q2)*sin(q3) - cos(q2)*cos(q3)*sin(q1))^2 - Iyy3*(cos(q2)*sin(q1)*sin(q3) + cos(q3)*sin(q1)*sin(q2))^2 - Izz3*cos(q1)^2 + Izz3*sin(q1)^2)))/2 + sin(q1)*(Ixx3*(cos(q1)*cos(q2)*sin(q3) + cos(q1)*cos(q3)*sin(q2))*(cos(q2)*sin(q3) + cos(q3)*sin(q2)) - Ixx3*(cos(q1)*cos(q2)*cos(q3) - cos(q1)*sin(q2)*sin(q3))*(cos(q2)*cos(q3) - sin(q2)*sin(q3)) - Iyy3*(cos(q1)*cos(q2)*sin(q3) + cos(q1)*cos(q3)*sin(q2))*(cos(q2)*sin(q3) + cos(q3)*sin(q2)) + Iyy3*(cos(q1)*cos(q2)*cos(q3) - cos(q1)*sin(q2)*sin(q3))*(cos(q2)*cos(q3) - sin(q2)*sin(q3))) - cos(q1)*(Ixx3*(cos(q2)*sin(q1)*sin(q3) + cos(q3)*sin(q1)*sin(q2))*(cos(q2)*sin(q3) + cos(q3)*sin(q2)) + Ixx3*(sin(q1)*sin(q2)*sin(q3) - cos(q2)*cos(q3)*sin(q1))*(cos(q2)*cos(q3) - sin(q2)*sin(q3)) - Iyy3*(cos(q2)*sin(q1)*sin(q3) + cos(q3)*sin(q1)*sin(q2))*(cos(q2)*sin(q3) + cos(q3)*sin(q2)) - Iyy3*(sin(q1)*sin(q2)*sin(q3) - cos(q2)*cos(q3)*sin(q1))*(cos(q2)*cos(q3) - sin(q2)*sin(q3))) + 2*m3*(lc3*cos(q2)*sin(q1)*sin(q3) + lc3*cos(q3)*sin(q1)*sin(q2))*(l2*cos(q1)*sin(q2) + lc3*cos(q1)*cos(q2)*sin(q3) + lc3*cos(q1)*cos(q3)*sin(q2)) - 2*m3*(lc3*cos(q1)*cos(q2)*cos(q3) - lc3*cos(q1)*sin(q2)*sin(q3))*(l2*cos(q2)*sin(q1) + lc3*cos(q2)*cos(q3)*sin(q1) - lc3*sin(q1)*sin(q2)*sin(q3)) + 2*m3*(lc3*cos(q1)*cos(q2)*sin(q3) + lc3*cos(q1)*cos(q3)*sin(q2))*(l2*sin(q1)*sin(q2) + lc3*cos(q2)*sin(q1)*sin(q3) + lc3*cos(q3)*sin(q1)*sin(q2))) + q1_d*(2*m3*(lc3*cos(q1)*cos(q2)*sin(q3) + lc3*cos(q1)*cos(q3)*sin(q2))*(l2*cos(q1)*cos(q2) + lc3*cos(q1)*cos(q2)*cos(q3) - lc3*cos(q1)*sin(q2)*sin(q3)) - 4*m3*(lc3*cos(q2)*sin(q1)*sin(q3) + lc3*cos(q3)*sin(q1)*sin(q2))*(l2*cos(q2)*sin(q1) + lc3*cos(q2)*cos(q3)*sin(q1) - lc3*sin(q1)*sin(q2)*sin(q3)) + Ixx3*(cos(q2)*sin(q3) + cos(q3)*sin(q2))*(cos(q2)*cos(q3) - sin(q2)*sin(q3)) - Iyy3*(cos(q2)*sin(q3) + cos(q3)*sin(q2))*(cos(q2)*cos(q3) - sin(q2)*sin(q3)));
     q1_d*(Iyy2*cos(q2)*sin(q2) - Ixx2*cos(q2)*sin(q2) - Ixx3*(cos(q2)*sin(q3) + cos(q3)*sin(q2))*(cos(q2)*cos(q3) - sin(q2)*sin(q3)) + Iyy3*(cos(q2)*sin(q3) + cos(q3)*sin(q2))*(cos(q2)*cos(q3) - sin(q2)*sin(q3)) + 2*m3*(l2*cos(q1)*cos(q2) + lc3*cos(q1)*cos(q2)*cos(q3) - lc3*cos(q1)*sin(q2)*sin(q3))*(l2*cos(q1)*sin(q2) + lc3*cos(q1)*cos(q2)*sin(q3) + lc3*cos(q1)*cos(q3)*sin(q2)) + lc2^2*m2*cos(q1)^2*cos(q2)*sin(q2) + lc2^2*m2*cos(q2)*sin(q1)^2*sin(q2)) - q3_d*((sin(q1)*(cos(q1)*(Ixx3*(sin(q1)*sin(q2)*sin(q3) - cos(q2)*cos(q3)*sin(q1))^2 + Iyy3*(cos(q2)*sin(q1)*sin(q3) + cos(q3)*sin(q1)*sin(q2))^2 + Izz3*cos(q1)^2) + sin(q1)*(Ixx3*(cos(q1)*cos(q2)*cos(q3) - cos(q1)*sin(q2)*sin(q3))*(sin(q1)*sin(q2)*sin(q3) - cos(q2)*cos(q3)*sin(q1)) - Iyy3*(cos(q1)*cos(q2)*sin(q3) + cos(q1)*cos(q3)*sin(q2))*(cos(q2)*sin(q1)*sin(q3) + cos(q3)*sin(q1)*sin(q2)) + Izz3*cos(q1)*sin(q1))))/2 - (sin(q1)*(cos(q1)*(Ixx3*(cos(q1)*cos(q2)*cos(q3) - cos(q1)*sin(q2)*sin(q3))^2 + Iyy3*(cos(q1)*cos(q2)*sin(q3) + cos(q1)*cos(q3)*sin(q2))^2 + Izz3*sin(q1)^2) - sin(q1)*(Ixx3*(cos(q1)*cos(q2)*cos(q3) - cos(q1)*sin(q2)*sin(q3))*(sin(q1)*sin(q2)*sin(q3) - cos(q2)*cos(q3)*sin(q1)) - Iyy3*(cos(q1)*cos(q2)*sin(q3) + cos(q1)*cos(q3)*sin(q2))*(cos(q2)*sin(q1)*sin(q3) + cos(q3)*sin(q1)*sin(q2)) + Izz3*cos(q1)*sin(q1)) + sin(q1)*(2*Ixx3*(cos(q1)*cos(q2)*cos(q3) - cos(q1)*sin(q2)*sin(q3))*(sin(q1)*sin(q2)*sin(q3) - cos(q2)*cos(q3)*sin(q1)) - 2*Iyy3*(cos(q1)*cos(q2)*sin(q3) + cos(q1)*cos(q3)*sin(q2))*(cos(q2)*sin(q1)*sin(q3) + cos(q3)*sin(q1)*sin(q2)) + 2*Izz3*cos(q1)*sin(q1)) - cos(q1)*(Ixx3*(cos(q1)*cos(q2)*cos(q3) - cos(q1)*sin(q2)*sin(q3))^2 + Iyy3*(cos(q1)*cos(q2)*sin(q3) + cos(q1)*cos(q3)*sin(q2))^2 - Ixx3*(sin(q1)*sin(q2)*sin(q3) - cos(q2)*cos(q3)*sin(q1))^2 - Iyy3*(cos(q2)*sin(q1)*sin(q3) + cos(q3)*sin(q1)*sin(q2))^2 - Izz3*cos(q1)^2 + Izz3*sin(q1)^2)))/2 - (cos(q1)*(sin(q1)*(Ixx3*(cos(q1)*cos(q2)*cos(q3) - cos(q1)*sin(q2)*sin(q3))^2 + Iyy3*(cos(q1)*cos(q2)*sin(q3) + cos(q1)*cos(q3)*sin(q2))^2 + Izz3*sin(q1)^2) + cos(q1)*(Ixx3*(cos(q1)*cos(q2)*cos(q3) - cos(q1)*sin(q2)*sin(q3))*(sin(q1)*sin(q2)*sin(q3) - cos(q2)*cos(q3)*sin(q1)) - Iyy3*(cos(q1)*cos(q2)*sin(q3) + cos(q1)*cos(q3)*sin(q2))*(cos(q2)*sin(q1)*sin(q3) + cos(q3)*sin(q1)*sin(q2)) + Izz3*cos(q1)*sin(q1))))/2 + (cos(q1)*(sin(q1)*(Ixx3*(sin(q1)*sin(q2)*sin(q3) - cos(q2)*cos(q3)*sin(q1))^2 + Iyy3*(cos(q2)*sin(q1)*sin(q3) + cos(q3)*sin(q1)*sin(q2))^2 + Izz3*cos(q1)^2) - cos(q1)*(Ixx3*(cos(q1)*cos(q2)*cos(q3) - cos(q1)*sin(q2)*sin(q3))*(sin(q1)*sin(q2)*sin(q3) - cos(q2)*cos(q3)*sin(q1)) - Iyy3*(cos(q1)*cos(q2)*sin(q3) + cos(q1)*cos(q3)*sin(q2))*(cos(q2)*sin(q1)*sin(q3) + cos(q3)*sin(q1)*sin(q2)) + Izz3*cos(q1)*sin(q1)) + cos(q1)*(2*Ixx3*(cos(q1)*cos(q2)*cos(q3) - cos(q1)*sin(q2)*sin(q3))*(sin(q1)*sin(q2)*sin(q3) - cos(q2)*cos(q3)*sin(q1)) - 2*Iyy3*(cos(q1)*cos(q2)*sin(q3) + cos(q1)*cos(q3)*sin(q2))*(cos(q2)*sin(q1)*sin(q3) + cos(q3)*sin(q1)*sin(q2)) + 2*Izz3*cos(q1)*sin(q1)) + sin(q1)*(Ixx3*(cos(q1)*cos(q2)*cos(q3) - cos(q1)*sin(q2)*sin(q3))^2 + Iyy3*(cos(q1)*cos(q2)*sin(q3) + cos(q1)*cos(q3)*sin(q2))^2 - Ixx3*(sin(q1)*sin(q2)*sin(q3) - cos(q2)*cos(q3)*sin(q1))^2 - Iyy3*(cos(q2)*sin(q1)*sin(q3) + cos(q3)*sin(q1)*sin(q2))^2 - Izz3*cos(q1)^2 + Izz3*sin(q1)^2)))/2 + 2*m3*(lc3*cos(q2)*sin(q1)*sin(q3) + lc3*cos(q3)*sin(q1)*sin(q2))*(l2*cos(q1)*sin(q2) + lc3*cos(q1)*cos(q2)*sin(q3) + lc3*cos(q1)*cos(q3)*sin(q2))) - q2_d*((sin(q1)*(cos(q1)*(Ixx3*(sin(q1)*sin(q2)*sin(q3) - cos(q2)*cos(q3)*sin(q1))^2 + Iyy3*(cos(q2)*sin(q1)*sin(q3) + cos(q3)*sin(q1)*sin(q2))^2 + Izz3*cos(q1)^2) + sin(q1)*(Ixx3*(cos(q1)*cos(q2)*cos(q3) - cos(q1)*sin(q2)*sin(q3))*(sin(q1)*sin(q2)*sin(q3) - cos(q2)*cos(q3)*sin(q1)) - Iyy3*(cos(q1)*cos(q2)*sin(q3) + cos(q1)*cos(q3)*sin(q2))*(cos(q2)*sin(q1)*sin(q3) + cos(q3)*sin(q1)*sin(q2)) + Izz3*cos(q1)*sin(q1))))/2 - (sin(q1)*(cos(q1)*(Ixx3*(cos(q1)*cos(q2)*cos(q3) - cos(q1)*sin(q2)*sin(q3))^2 + Iyy3*(cos(q1)*cos(q2)*sin(q3) + cos(q1)*cos(q3)*sin(q2))^2 + Izz3*sin(q1)^2) - sin(q1)*(Ixx3*(cos(q1)*cos(q2)*cos(q3) - cos(q1)*sin(q2)*sin(q3))*(sin(q1)*sin(q2)*sin(q3) - cos(q2)*cos(q3)*sin(q1)) - Iyy3*(cos(q1)*cos(q2)*sin(q3) + cos(q1)*cos(q3)*sin(q2))*(cos(q2)*sin(q1)*sin(q3) + cos(q3)*sin(q1)*sin(q2)) + Izz3*cos(q1)*sin(q1)) + sin(q1)*(2*Ixx3*(cos(q1)*cos(q2)*cos(q3) - cos(q1)*sin(q2)*sin(q3))*(sin(q1)*sin(q2)*sin(q3) - cos(q2)*cos(q3)*sin(q1)) - 2*Iyy3*(cos(q1)*cos(q2)*sin(q3) + cos(q1)*cos(q3)*sin(q2))*(cos(q2)*sin(q1)*sin(q3) + cos(q3)*sin(q1)*sin(q2)) + 2*Izz3*cos(q1)*sin(q1)) - cos(q1)*(Ixx3*(cos(q1)*cos(q2)*cos(q3) - cos(q1)*sin(q2)*sin(q3))^2 + Iyy3*(cos(q1)*cos(q2)*sin(q3) + cos(q1)*cos(q3)*sin(q2))^2 - Ixx3*(sin(q1)*sin(q2)*sin(q3) - cos(q2)*cos(q3)*sin(q1))^2 - Iyy3*(cos(q2)*sin(q1)*sin(q3) + cos(q3)*sin(q1)*sin(q2))^2 - Izz3*cos(q1)^2 + Izz3*sin(q1)^2)))/2 - (cos(q1)*(sin(q1)*(Ixx3*(cos(q1)*cos(q2)*cos(q3) - cos(q1)*sin(q2)*sin(q3))^2 + Iyy3*(cos(q1)*cos(q2)*sin(q3) + cos(q1)*cos(q3)*sin(q2))^2 + Izz3*sin(q1)^2) + cos(q1)*(Ixx3*(cos(q1)*cos(q2)*cos(q3) - cos(q1)*sin(q2)*sin(q3))*(sin(q1)*sin(q2)*sin(q3) - cos(q2)*cos(q3)*sin(q1)) - Iyy3*(cos(q1)*cos(q2)*sin(q3) + cos(q1)*cos(q3)*sin(q2))*(cos(q2)*sin(q1)*sin(q3) + cos(q3)*sin(q1)*sin(q2)) + Izz3*cos(q1)*sin(q1))))/2 + (cos(q1)*(sin(q1)*(Ixx3*(sin(q1)*sin(q2)*sin(q3) - cos(q2)*cos(q3)*sin(q1))^2 + Iyy3*(cos(q2)*sin(q1)*sin(q3) + cos(q3)*sin(q1)*sin(q2))^2 + Izz3*cos(q1)^2) - cos(q1)*(Ixx3*(cos(q1)*cos(q2)*cos(q3) - cos(q1)*sin(q2)*sin(q3))*(sin(q1)*sin(q2)*sin(q3) - cos(q2)*cos(q3)*sin(q1)) - Iyy3*(cos(q1)*cos(q2)*sin(q3) + cos(q1)*cos(q3)*sin(q2))*(cos(q2)*sin(q1)*sin(q3) + cos(q3)*sin(q1)*sin(q2)) + Izz3*cos(q1)*sin(q1)) + cos(q1)*(2*Ixx3*(cos(q1)*cos(q2)*cos(q3) - cos(q1)*sin(q2)*sin(q3))*(sin(q1)*sin(q2)*sin(q3) - cos(q2)*cos(q3)*sin(q1)) - 2*Iyy3*(cos(q1)*cos(q2)*sin(q3) + cos(q1)*cos(q3)*sin(q2))*(cos(q2)*sin(q1)*sin(q3) + cos(q3)*sin(q1)*sin(q2)) + 2*Izz3*cos(q1)*sin(q1)) + sin(q1)*(Ixx3*(cos(q1)*cos(q2)*cos(q3) - cos(q1)*sin(q2)*sin(q3))^2 + Iyy3*(cos(q1)*cos(q2)*sin(q3) + cos(q1)*cos(q3)*sin(q2))^2 - Ixx3*(sin(q1)*sin(q2)*sin(q3) - cos(q2)*cos(q3)*sin(q1))^2 - Iyy3*(cos(q2)*sin(q1)*sin(q3) + cos(q3)*sin(q1)*sin(q2))^2 - Izz3*cos(q1)^2 + Izz3*sin(q1)^2)))/2 + (cos(q1)*(cos(q1)*(Ixx2*cos(q1)*cos(q2)^2*sin(q1) - Izz2*cos(q1)*sin(q1) + Iyy2*cos(q1)*sin(q1)*sin(q2)^2) - sin(q1)*(Ixx2*cos(q1)^2*cos(q2)^2 + Iyy2*cos(q1)^2*sin(q2)^2 + Izz2*sin(q1)^2)))/2 - (sin(q1)*(sin(q1)*(Ixx2*cos(q1)*cos(q2)^2*sin(q1) - Izz2*cos(q1)*sin(q1) + Iyy2*cos(q1)*sin(q1)*sin(q2)^2) - cos(q1)*(Izz2*cos(q1)^2 + Ixx2*cos(q2)^2*sin(q1)^2 + Iyy2*sin(q1)^2*sin(q2)^2)))/2 - (sin(q1)*(sin(q1)*(Ixx2*cos(q1)*cos(q2)^2*sin(q1) - Izz2*cos(q1)*sin(q1) + Iyy2*cos(q1)*sin(q1)*sin(q2)^2) - sin(q1)*(2*Ixx2*cos(q1)*cos(q2)^2*sin(q1) - 2*Izz2*cos(q1)*sin(q1) + 2*Iyy2*cos(q1)*sin(q1)*sin(q2)^2) + cos(q1)*(Ixx2*cos(q1)^2*cos(q2)^2 + Iyy2*cos(q1)^2*sin(q2)^2 + Izz2*sin(q1)^2) + cos(q1)*(- Ixx2*cos(q1)^2*cos(q2)^2 - Iyy2*cos(q1)^2*sin(q2)^2 + Izz2*cos(q1)^2 + Ixx2*cos(q2)^2*sin(q1)^2 + Iyy2*sin(q1)^2*sin(q2)^2 - Izz2*sin(q1)^2)))/2 + (cos(q1)*(cos(q1)*(Ixx2*cos(q1)*cos(q2)^2*sin(q1) - Izz2*cos(q1)*sin(q1) + Iyy2*cos(q1)*sin(q1)*sin(q2)^2) - cos(q1)*(2*Ixx2*cos(q1)*cos(q2)^2*sin(q1) - 2*Izz2*cos(q1)*sin(q1) + 2*Iyy2*cos(q1)*sin(q1)*sin(q2)^2) + sin(q1)*(Izz2*cos(q1)^2 + Ixx2*cos(q2)^2*sin(q1)^2 + Iyy2*sin(q1)^2*sin(q2)^2) - sin(q1)*(- Ixx2*cos(q1)^2*cos(q2)^2 - Iyy2*cos(q1)^2*sin(q2)^2 + Izz2*cos(q1)^2 + Ixx2*cos(q2)^2*sin(q1)^2 + Iyy2*sin(q1)^2*sin(q2)^2 - Izz2*sin(q1)^2)))/2 + 2*m3*(l2*cos(q1)*sin(q2) + lc3*cos(q1)*cos(q2)*sin(q3) + lc3*cos(q1)*cos(q3)*sin(q2))*(l2*sin(q1)*sin(q2) + lc3*cos(q2)*sin(q1)*sin(q3) + lc3*cos(q3)*sin(q1)*sin(q2))), q3_d*((cos(q1)*(cos(q1)*(2*Ixx3*(cos(q2)*sin(q1)*sin(q3) + cos(q3)*sin(q1)*sin(q2))*(sin(q1)*sin(q2)*sin(q3) - cos(q2)*cos(q3)*sin(q1)) - 2*Iyy3*(cos(q2)*sin(q1)*sin(q3) + cos(q3)*sin(q1)*sin(q2))*(sin(q1)*sin(q2)*sin(q3) - cos(q2)*cos(q3)*sin(q1))) - sin(q1)*(Ixx3*(cos(q1)*cos(q2)*sin(q3) + cos(q1)*cos(q3)*sin(q2))*(sin(q1)*sin(q2)*sin(q3) - cos(q2)*cos(q3)*sin(q1)) - Ixx3*(cos(q1)*cos(q2)*cos(q3) - cos(q1)*sin(q2)*sin(q3))*(cos(q2)*sin(q1)*sin(q3) + cos(q3)*sin(q1)*sin(q2)) - Iyy3*(cos(q1)*cos(q2)*sin(q3) + cos(q1)*cos(q3)*sin(q2))*(sin(q1)*sin(q2)*sin(q3) - cos(q2)*cos(q3)*sin(q1)) + Iyy3*(cos(q1)*cos(q2)*cos(q3) - cos(q1)*sin(q2)*sin(q3))*(cos(q2)*sin(q1)*sin(q3) + cos(q3)*sin(q1)*sin(q2)))))/2 - (sin(q1)*(cos(q1)*(Ixx3*(cos(q1)*cos(q2)*sin(q3) + cos(q1)*cos(q3)*sin(q2))*(sin(q1)*sin(q2)*sin(q3) - cos(q2)*cos(q3)*sin(q1)) - Ixx3*(cos(q1)*cos(q2)*cos(q3) - cos(q1)*sin(q2)*sin(q3))*(cos(q2)*sin(q1)*sin(q3) + cos(q3)*sin(q1)*sin(q2)) - Iyy3*(cos(q1)*cos(q2)*sin(q3) + cos(q1)*cos(q3)*sin(q2))*(sin(q1)*sin(q2)*sin(q3) - cos(q2)*cos(q3)*sin(q1)) + Iyy3*(cos(q1)*cos(q2)*cos(q3) - cos(q1)*sin(q2)*sin(q3))*(cos(q2)*sin(q1)*sin(q3) + cos(q3)*sin(q1)*sin(q2))) + sin(q1)*(2*Ixx3*(cos(q1)*cos(q2)*sin(q3) + cos(q1)*cos(q3)*sin(q2))*(cos(q1)*cos(q2)*cos(q3) - cos(q1)*sin(q2)*sin(q3)) - 2*Iyy3*(cos(q1)*cos(q2)*sin(q3) + cos(q1)*cos(q3)*sin(q2))*(cos(q1)*cos(q2)*cos(q3) - cos(q1)*sin(q2)*sin(q3)))))/2 - m3*(lc3*cos(q2)*sin(q3) + lc3*cos(q3)*sin(q2))*(cos(q2)*(l1 + l2) + lc3*cos(q2)*cos(q3) - lc3*sin(q2)*sin(q3)) + 2*m3*(lc3*cos(q1)*cos(q2)*cos(q3) - lc3*cos(q1)*sin(q2)*sin(q3))*(l2*cos(q1)*sin(q2) + lc3*cos(q1)*cos(q2)*sin(q3) + lc3*cos(q1)*cos(q3)*sin(q2))) + q2_d*((sin(q1)*(cos(q1)*(2*Ixx2*cos(q1)*cos(q2)*sin(q1)*sin(q2) - 2*Iyy2*cos(q1)*cos(q2)*sin(q1)*sin(q2)) - sin(q1)*(2*Ixx2*cos(q1)^2*cos(q2)*sin(q2) - 2*Iyy2*cos(q1)^2*cos(q2)*sin(q2))))/2 + (cos(q1)*(sin(q1)*(2*Ixx2*cos(q1)*cos(q2)*sin(q1)*sin(q2) - 2*Iyy2*cos(q1)*cos(q2)*sin(q1)*sin(q2)) - cos(q1)*(2*Ixx2*cos(q2)*sin(q1)^2*sin(q2) - 2*Iyy2*cos(q2)*sin(q1)^2*sin(q2))))/2 + (cos(q1)*(cos(q1)*(2*Ixx3*(cos(q2)*sin(q1)*sin(q3) + cos(q3)*sin(q1)*sin(q2))*(sin(q1)*sin(q2)*sin(q3) - cos(q2)*cos(q3)*sin(q1)) - 2*Iyy3*(cos(q2)*sin(q1)*sin(q3) + cos(q3)*sin(q1)*sin(q2))*(sin(q1)*sin(q2)*sin(q3) - cos(q2)*cos(q3)*sin(q1))) - sin(q1)*(Ixx3*(cos(q1)*cos(q2)*sin(q3) + cos(q1)*cos(q3)*sin(q2))*(sin(q1)*sin(q2)*sin(q3) - cos(q2)*cos(q3)*sin(q1)) - Ixx3*(cos(q1)*cos(q2)*cos(q3) - cos(q1)*sin(q2)*sin(q3))*(cos(q2)*sin(q1)*sin(q3) + cos(q3)*sin(q1)*sin(q2)) - Iyy3*(cos(q1)*cos(q2)*sin(q3) + cos(q1)*cos(q3)*sin(q2))*(sin(q1)*sin(q2)*sin(q3) - cos(q2)*cos(q3)*sin(q1)) + Iyy3*(cos(q1)*cos(q2)*cos(q3) - cos(q1)*sin(q2)*sin(q3))*(cos(q2)*sin(q1)*sin(q3) + cos(q3)*sin(q1)*sin(q2)))))/2 - (sin(q1)*(cos(q1)*(Ixx3*(cos(q1)*cos(q2)*sin(q3) + cos(q1)*cos(q3)*sin(q2))*(sin(q1)*sin(q2)*sin(q3) - cos(q2)*cos(q3)*sin(q1)) - Ixx3*(cos(q1)*cos(q2)*cos(q3) - cos(q1)*sin(q2)*sin(q3))*(cos(q2)*sin(q1)*sin(q3) + cos(q3)*sin(q1)*sin(q2)) - Iyy3*(cos(q1)*cos(q2)*sin(q3) + cos(q1)*cos(q3)*sin(q2))*(sin(q1)*sin(q2)*sin(q3) - cos(q2)*cos(q3)*sin(q1)) + Iyy3*(cos(q1)*cos(q2)*cos(q3) - cos(q1)*sin(q2)*sin(q3))*(cos(q2)*sin(q1)*sin(q3) + cos(q3)*sin(q1)*sin(q2))) + sin(q1)*(2*Ixx3*(cos(q1)*cos(q2)*sin(q3) + cos(q1)*cos(q3)*sin(q2))*(cos(q1)*cos(q2)*cos(q3) - cos(q1)*sin(q2)*sin(q3)) - 2*Iyy3*(cos(q1)*cos(q2)*sin(q3) + cos(q1)*cos(q3)*sin(q2))*(cos(q1)*cos(q2)*cos(q3) - cos(q1)*sin(q2)*sin(q3)))))/2 - m3*(cos(q2)*(l1 + l2) + lc3*cos(q2)*cos(q3) - lc3*sin(q2)*sin(q3))*(sin(q2)*(l1 + l2) + lc3*cos(q2)*sin(q3) + lc3*cos(q3)*sin(q2)) + 2*m3*(l2*cos(q1)*cos(q2) + lc3*cos(q1)*cos(q2)*cos(q3) - lc3*cos(q1)*sin(q2)*sin(q3))*(l2*cos(q1)*sin(q2) + lc3*cos(q1)*cos(q2)*sin(q3) + lc3*cos(q1)*cos(q3)*sin(q2)) - m2*cos(q2)*sin(q2)*(l1 + lc2)^2 + lc2^2*m2*cos(q1)^2*cos(q2)*sin(q2) + lc2^2*m2*cos(q2)*sin(q1)^2*sin(q2)) - q1_d*((sin(q1)*(cos(q1)*(Ixx3*(sin(q1)*sin(q2)*sin(q3) - cos(q2)*cos(q3)*sin(q1))^2 + Iyy3*(cos(q2)*sin(q1)*sin(q3) + cos(q3)*sin(q1)*sin(q2))^2 + Izz3*cos(q1)^2) + sin(q1)*(Ixx3*(cos(q1)*cos(q2)*cos(q3) - cos(q1)*sin(q2)*sin(q3))*(sin(q1)*sin(q2)*sin(q3) - cos(q2)*cos(q3)*sin(q1)) - Iyy3*(cos(q1)*cos(q2)*sin(q3) + cos(q1)*cos(q3)*sin(q2))*(cos(q2)*sin(q1)*sin(q3) + cos(q3)*sin(q1)*sin(q2)) + Izz3*cos(q1)*sin(q1))))/2 - (sin(q1)*(cos(q1)*(Ixx3*(cos(q1)*cos(q2)*cos(q3) - cos(q1)*sin(q2)*sin(q3))^2 + Iyy3*(cos(q1)*cos(q2)*sin(q3) + cos(q1)*cos(q3)*sin(q2))^2 + Izz3*sin(q1)^2) - sin(q1)*(Ixx3*(cos(q1)*cos(q2)*cos(q3) - cos(q1)*sin(q2)*sin(q3))*(sin(q1)*sin(q2)*sin(q3) - cos(q2)*cos(q3)*sin(q1)) - Iyy3*(cos(q1)*cos(q2)*sin(q3) + cos(q1)*cos(q3)*sin(q2))*(cos(q2)*sin(q1)*sin(q3) + cos(q3)*sin(q1)*sin(q2)) + Izz3*cos(q1)*sin(q1)) + sin(q1)*(2*Ixx3*(cos(q1)*cos(q2)*cos(q3) - cos(q1)*sin(q2)*sin(q3))*(sin(q1)*sin(q2)*sin(q3) - cos(q2)*cos(q3)*sin(q1)) - 2*Iyy3*(cos(q1)*cos(q2)*sin(q3) + cos(q1)*cos(q3)*sin(q2))*(cos(q2)*sin(q1)*sin(q3) + cos(q3)*sin(q1)*sin(q2)) + 2*Izz3*cos(q1)*sin(q1)) - cos(q1)*(Ixx3*(cos(q1)*cos(q2)*cos(q3) - cos(q1)*sin(q2)*sin(q3))^2 + Iyy3*(cos(q1)*cos(q2)*sin(q3) + cos(q1)*cos(q3)*sin(q2))^2 - Ixx3*(sin(q1)*sin(q2)*sin(q3) - cos(q2)*cos(q3)*sin(q1))^2 - Iyy3*(cos(q2)*sin(q1)*sin(q3) + cos(q3)*sin(q1)*sin(q2))^2 - Izz3*cos(q1)^2 + Izz3*sin(q1)^2)))/2 - (cos(q1)*(sin(q1)*(Ixx3*(cos(q1)*cos(q2)*cos(q3) - cos(q1)*sin(q2)*sin(q3))^2 + Iyy3*(cos(q1)*cos(q2)*sin(q3) + cos(q1)*cos(q3)*sin(q2))^2 + Izz3*sin(q1)^2) + cos(q1)*(Ixx3*(cos(q1)*cos(q2)*cos(q3) - cos(q1)*sin(q2)*sin(q3))*(sin(q1)*sin(q2)*sin(q3) - cos(q2)*cos(q3)*sin(q1)) - Iyy3*(cos(q1)*cos(q2)*sin(q3) + cos(q1)*cos(q3)*sin(q2))*(cos(q2)*sin(q1)*sin(q3) + cos(q3)*sin(q1)*sin(q2)) + Izz3*cos(q1)*sin(q1))))/2 + (cos(q1)*(sin(q1)*(Ixx3*(sin(q1)*sin(q2)*sin(q3) - cos(q2)*cos(q3)*sin(q1))^2 + Iyy3*(cos(q2)*sin(q1)*sin(q3) + cos(q3)*sin(q1)*sin(q2))^2 + Izz3*cos(q1)^2) - cos(q1)*(Ixx3*(cos(q1)*cos(q2)*cos(q3) - cos(q1)*sin(q2)*sin(q3))*(sin(q1)*sin(q2)*sin(q3) - cos(q2)*cos(q3)*sin(q1)) - Iyy3*(cos(q1)*cos(q2)*sin(q3) + cos(q1)*cos(q3)*sin(q2))*(cos(q2)*sin(q1)*sin(q3) + cos(q3)*sin(q1)*sin(q2)) + Izz3*cos(q1)*sin(q1)) + cos(q1)*(2*Ixx3*(cos(q1)*cos(q2)*cos(q3) - cos(q1)*sin(q2)*sin(q3))*(sin(q1)*sin(q2)*sin(q3) - cos(q2)*cos(q3)*sin(q1)) - 2*Iyy3*(cos(q1)*cos(q2)*sin(q3) + cos(q1)*cos(q3)*sin(q2))*(cos(q2)*sin(q1)*sin(q3) + cos(q3)*sin(q1)*sin(q2)) + 2*Izz3*cos(q1)*sin(q1)) + sin(q1)*(Ixx3*(cos(q1)*cos(q2)*cos(q3) - cos(q1)*sin(q2)*sin(q3))^2 + Iyy3*(cos(q1)*cos(q2)*sin(q3) + cos(q1)*cos(q3)*sin(q2))^2 - Ixx3*(sin(q1)*sin(q2)*sin(q3) - cos(q2)*cos(q3)*sin(q1))^2 - Iyy3*(cos(q2)*sin(q1)*sin(q3) + cos(q3)*sin(q1)*sin(q2))^2 - Izz3*cos(q1)^2 + Izz3*sin(q1)^2)))/2 + (cos(q1)*(cos(q1)*(Ixx2*cos(q1)*cos(q2)^2*sin(q1) - Izz2*cos(q1)*sin(q1) + Iyy2*cos(q1)*sin(q1)*sin(q2)^2) - sin(q1)*(Ixx2*cos(q1)^2*cos(q2)^2 + Iyy2*cos(q1)^2*sin(q2)^2 + Izz2*sin(q1)^2)))/2 - (sin(q1)*(sin(q1)*(Ixx2*cos(q1)*cos(q2)^2*sin(q1) - Izz2*cos(q1)*sin(q1) + Iyy2*cos(q1)*sin(q1)*sin(q2)^2) - cos(q1)*(Izz2*cos(q1)^2 + Ixx2*cos(q2)^2*sin(q1)^2 + Iyy2*sin(q1)^2*sin(q2)^2)))/2 - (sin(q1)*(sin(q1)*(Ixx2*cos(q1)*cos(q2)^2*sin(q1) - Izz2*cos(q1)*sin(q1) + Iyy2*cos(q1)*sin(q1)*sin(q2)^2) - sin(q1)*(2*Ixx2*cos(q1)*cos(q2)^2*sin(q1) - 2*Izz2*cos(q1)*sin(q1) + 2*Iyy2*cos(q1)*sin(q1)*sin(q2)^2) + cos(q1)*(Ixx2*cos(q1)^2*cos(q2)^2 + Iyy2*cos(q1)^2*sin(q2)^2 + Izz2*sin(q1)^2) + cos(q1)*(- Ixx2*cos(q1)^2*cos(q2)^2 - Iyy2*cos(q1)^2*sin(q2)^2 + Izz2*cos(q1)^2 + Ixx2*cos(q2)^2*sin(q1)^2 + Iyy2*sin(q1)^2*sin(q2)^2 - Izz2*sin(q1)^2)))/2 + (cos(q1)*(cos(q1)*(Ixx2*cos(q1)*cos(q2)^2*sin(q1) - Izz2*cos(q1)*sin(q1) + Iyy2*cos(q1)*sin(q1)*sin(q2)^2) - cos(q1)*(2*Ixx2*cos(q1)*cos(q2)^2*sin(q1) - 2*Izz2*cos(q1)*sin(q1) + 2*Iyy2*cos(q1)*sin(q1)*sin(q2)^2) + sin(q1)*(Izz2*cos(q1)^2 + Ixx2*cos(q2)^2*sin(q1)^2 + Iyy2*sin(q1)^2*sin(q2)^2) - sin(q1)*(- Ixx2*cos(q1)^2*cos(q2)^2 - Iyy2*cos(q1)^2*sin(q2)^2 + Izz2*cos(q1)^2 + Ixx2*cos(q2)^2*sin(q1)^2 + Iyy2*sin(q1)^2*sin(q2)^2 - Izz2*sin(q1)^2)))/2 + 2*m3*(l2*cos(q1)*sin(q2) + lc3*cos(q1)*cos(q2)*sin(q3) + lc3*cos(q1)*cos(q3)*sin(q2))*(l2*sin(q1)*sin(q2) + lc3*cos(q2)*sin(q1)*sin(q3) + lc3*cos(q3)*sin(q1)*sin(q2))), q2_d*((cos(q1)*(cos(q1)*(2*Ixx3*(cos(q2)*sin(q1)*sin(q3) + cos(q3)*sin(q1)*sin(q2))*(sin(q1)*sin(q2)*sin(q3) - cos(q2)*cos(q3)*sin(q1)) - 2*Iyy3*(cos(q2)*sin(q1)*sin(q3) + cos(q3)*sin(q1)*sin(q2))*(sin(q1)*sin(q2)*sin(q3) - cos(q2)*cos(q3)*sin(q1))) - sin(q1)*(Ixx3*(cos(q1)*cos(q2)*sin(q3) + cos(q1)*cos(q3)*sin(q2))*(sin(q1)*sin(q2)*sin(q3) - cos(q2)*cos(q3)*sin(q1)) - Ixx3*(cos(q1)*cos(q2)*cos(q3) - cos(q1)*sin(q2)*sin(q3))*(cos(q2)*sin(q1)*sin(q3) + cos(q3)*sin(q1)*sin(q2)) - Iyy3*(cos(q1)*cos(q2)*sin(q3) + cos(q1)*cos(q3)*sin(q2))*(sin(q1)*sin(q2)*sin(q3) - cos(q2)*cos(q3)*sin(q1)) + Iyy3*(cos(q1)*cos(q2)*cos(q3) - cos(q1)*sin(q2)*sin(q3))*(cos(q2)*sin(q1)*sin(q3) + cos(q3)*sin(q1)*sin(q2)))))/2 - (sin(q1)*(cos(q1)*(Ixx3*(cos(q1)*cos(q2)*sin(q3) + cos(q1)*cos(q3)*sin(q2))*(sin(q1)*sin(q2)*sin(q3) - cos(q2)*cos(q3)*sin(q1)) - Ixx3*(cos(q1)*cos(q2)*cos(q3) - cos(q1)*sin(q2)*sin(q3))*(cos(q2)*sin(q1)*sin(q3) + cos(q3)*sin(q1)*sin(q2)) - Iyy3*(cos(q1)*cos(q2)*sin(q3) + cos(q1)*cos(q3)*sin(q2))*(sin(q1)*sin(q2)*sin(q3) - cos(q2)*cos(q3)*sin(q1)) + Iyy3*(cos(q1)*cos(q2)*cos(q3) - cos(q1)*sin(q2)*sin(q3))*(cos(q2)*sin(q1)*sin(q3) + cos(q3)*sin(q1)*sin(q2))) + sin(q1)*(2*Ixx3*(cos(q1)*cos(q2)*sin(q3) + cos(q1)*cos(q3)*sin(q2))*(cos(q1)*cos(q2)*cos(q3) - cos(q1)*sin(q2)*sin(q3)) - 2*Iyy3*(cos(q1)*cos(q2)*sin(q3) + cos(q1)*cos(q3)*sin(q2))*(cos(q1)*cos(q2)*cos(q3) - cos(q1)*sin(q2)*sin(q3)))))/2 - m3*(lc3*cos(q2)*sin(q3) + lc3*cos(q3)*sin(q2))*(cos(q2)*(l1 + l2) + lc3*cos(q2)*cos(q3) - lc3*sin(q2)*sin(q3)) + 2*m3*(lc3*cos(q1)*cos(q2)*cos(q3) - lc3*cos(q1)*sin(q2)*sin(q3))*(l2*cos(q1)*sin(q2) + lc3*cos(q1)*cos(q2)*sin(q3) + lc3*cos(q1)*cos(q3)*sin(q2))) + q3_d*((cos(q1)*(cos(q1)*(2*Ixx3*(cos(q2)*sin(q1)*sin(q3) + cos(q3)*sin(q1)*sin(q2))*(sin(q1)*sin(q2)*sin(q3) - cos(q2)*cos(q3)*sin(q1)) - 2*Iyy3*(cos(q2)*sin(q1)*sin(q3) + cos(q3)*sin(q1)*sin(q2))*(sin(q1)*sin(q2)*sin(q3) - cos(q2)*cos(q3)*sin(q1))) - sin(q1)*(Ixx3*(cos(q1)*cos(q2)*sin(q3) + cos(q1)*cos(q3)*sin(q2))*(sin(q1)*sin(q2)*sin(q3) - cos(q2)*cos(q3)*sin(q1)) - Ixx3*(cos(q1)*cos(q2)*cos(q3) - cos(q1)*sin(q2)*sin(q3))*(cos(q2)*sin(q1)*sin(q3) + cos(q3)*sin(q1)*sin(q2)) - Iyy3*(cos(q1)*cos(q2)*sin(q3) + cos(q1)*cos(q3)*sin(q2))*(sin(q1)*sin(q2)*sin(q3) - cos(q2)*cos(q3)*sin(q1)) + Iyy3*(cos(q1)*cos(q2)*cos(q3) - cos(q1)*sin(q2)*sin(q3))*(cos(q2)*sin(q1)*sin(q3) + cos(q3)*sin(q1)*sin(q2)))))/2 - (sin(q1)*(cos(q1)*(Ixx3*(cos(q1)*cos(q2)*sin(q3) + cos(q1)*cos(q3)*sin(q2))*(sin(q1)*sin(q2)*sin(q3) - cos(q2)*cos(q3)*sin(q1)) - Ixx3*(cos(q1)*cos(q2)*cos(q3) - cos(q1)*sin(q2)*sin(q3))*(cos(q2)*sin(q1)*sin(q3) + cos(q3)*sin(q1)*sin(q2)) - Iyy3*(cos(q1)*cos(q2)*sin(q3) + cos(q1)*cos(q3)*sin(q2))*(sin(q1)*sin(q2)*sin(q3) - cos(q2)*cos(q3)*sin(q1)) + Iyy3*(cos(q1)*cos(q2)*cos(q3) - cos(q1)*sin(q2)*sin(q3))*(cos(q2)*sin(q1)*sin(q3) + cos(q3)*sin(q1)*sin(q2))) + sin(q1)*(2*Ixx3*(cos(q1)*cos(q2)*sin(q3) + cos(q1)*cos(q3)*sin(q2))*(cos(q1)*cos(q2)*cos(q3) - cos(q1)*sin(q2)*sin(q3)) - 2*Iyy3*(cos(q1)*cos(q2)*sin(q3) + cos(q1)*cos(q3)*sin(q2))*(cos(q1)*cos(q2)*cos(q3) - cos(q1)*sin(q2)*sin(q3)))))/2 - m3*(lc3*cos(q2)*sin(q3) + lc3*cos(q3)*sin(q2))*(cos(q2)*(l1 + l2) + lc3*cos(q2)*cos(q3) - lc3*sin(q2)*sin(q3)) + 2*m3*(lc3*cos(q1)*cos(q2)*cos(q3) - lc3*cos(q1)*sin(q2)*sin(q3))*(l2*cos(q1)*sin(q2) + lc3*cos(q1)*cos(q2)*sin(q3) + lc3*cos(q1)*cos(q3)*sin(q2))) - q1_d*((sin(q1)*(cos(q1)*(Ixx3*(sin(q1)*sin(q2)*sin(q3) - cos(q2)*cos(q3)*sin(q1))^2 + Iyy3*(cos(q2)*sin(q1)*sin(q3) + cos(q3)*sin(q1)*sin(q2))^2 + Izz3*cos(q1)^2) + sin(q1)*(Ixx3*(cos(q1)*cos(q2)*cos(q3) - cos(q1)*sin(q2)*sin(q3))*(sin(q1)*sin(q2)*sin(q3) - cos(q2)*cos(q3)*sin(q1)) - Iyy3*(cos(q1)*cos(q2)*sin(q3) + cos(q1)*cos(q3)*sin(q2))*(cos(q2)*sin(q1)*sin(q3) + cos(q3)*sin(q1)*sin(q2)) + Izz3*cos(q1)*sin(q1))))/2 - (sin(q1)*(cos(q1)*(Ixx3*(cos(q1)*cos(q2)*cos(q3) - cos(q1)*sin(q2)*sin(q3))^2 + Iyy3*(cos(q1)*cos(q2)*sin(q3) + cos(q1)*cos(q3)*sin(q2))^2 + Izz3*sin(q1)^2) - sin(q1)*(Ixx3*(cos(q1)*cos(q2)*cos(q3) - cos(q1)*sin(q2)*sin(q3))*(sin(q1)*sin(q2)*sin(q3) - cos(q2)*cos(q3)*sin(q1)) - Iyy3*(cos(q1)*cos(q2)*sin(q3) + cos(q1)*cos(q3)*sin(q2))*(cos(q2)*sin(q1)*sin(q3) + cos(q3)*sin(q1)*sin(q2)) + Izz3*cos(q1)*sin(q1)) + sin(q1)*(2*Ixx3*(cos(q1)*cos(q2)*cos(q3) - cos(q1)*sin(q2)*sin(q3))*(sin(q1)*sin(q2)*sin(q3) - cos(q2)*cos(q3)*sin(q1)) - 2*Iyy3*(cos(q1)*cos(q2)*sin(q3) + cos(q1)*cos(q3)*sin(q2))*(cos(q2)*sin(q1)*sin(q3) + cos(q3)*sin(q1)*sin(q2)) + 2*Izz3*cos(q1)*sin(q1)) - cos(q1)*(Ixx3*(cos(q1)*cos(q2)*cos(q3) - cos(q1)*sin(q2)*sin(q3))^2 + Iyy3*(cos(q1)*cos(q2)*sin(q3) + cos(q1)*cos(q3)*sin(q2))^2 - Ixx3*(sin(q1)*sin(q2)*sin(q3) - cos(q2)*cos(q3)*sin(q1))^2 - Iyy3*(cos(q2)*sin(q1)*sin(q3) + cos(q3)*sin(q1)*sin(q2))^2 - Izz3*cos(q1)^2 + Izz3*sin(q1)^2)))/2 - (cos(q1)*(sin(q1)*(Ixx3*(cos(q1)*cos(q2)*cos(q3) - cos(q1)*sin(q2)*sin(q3))^2 + Iyy3*(cos(q1)*cos(q2)*sin(q3) + cos(q1)*cos(q3)*sin(q2))^2 + Izz3*sin(q1)^2) + cos(q1)*(Ixx3*(cos(q1)*cos(q2)*cos(q3) - cos(q1)*sin(q2)*sin(q3))*(sin(q1)*sin(q2)*sin(q3) - cos(q2)*cos(q3)*sin(q1)) - Iyy3*(cos(q1)*cos(q2)*sin(q3) + cos(q1)*cos(q3)*sin(q2))*(cos(q2)*sin(q1)*sin(q3) + cos(q3)*sin(q1)*sin(q2)) + Izz3*cos(q1)*sin(q1))))/2 + (cos(q1)*(sin(q1)*(Ixx3*(sin(q1)*sin(q2)*sin(q3) - cos(q2)*cos(q3)*sin(q1))^2 + Iyy3*(cos(q2)*sin(q1)*sin(q3) + cos(q3)*sin(q1)*sin(q2))^2 + Izz3*cos(q1)^2) - cos(q1)*(Ixx3*(cos(q1)*cos(q2)*cos(q3) - cos(q1)*sin(q2)*sin(q3))*(sin(q1)*sin(q2)*sin(q3) - cos(q2)*cos(q3)*sin(q1)) - Iyy3*(cos(q1)*cos(q2)*sin(q3) + cos(q1)*cos(q3)*sin(q2))*(cos(q2)*sin(q1)*sin(q3) + cos(q3)*sin(q1)*sin(q2)) + Izz3*cos(q1)*sin(q1)) + cos(q1)*(2*Ixx3*(cos(q1)*cos(q2)*cos(q3) - cos(q1)*sin(q2)*sin(q3))*(sin(q1)*sin(q2)*sin(q3) - cos(q2)*cos(q3)*sin(q1)) - 2*Iyy3*(cos(q1)*cos(q2)*sin(q3) + cos(q1)*cos(q3)*sin(q2))*(cos(q2)*sin(q1)*sin(q3) + cos(q3)*sin(q1)*sin(q2)) + 2*Izz3*cos(q1)*sin(q1)) + sin(q1)*(Ixx3*(cos(q1)*cos(q2)*cos(q3) - cos(q1)*sin(q2)*sin(q3))^2 + Iyy3*(cos(q1)*cos(q2)*sin(q3) + cos(q1)*cos(q3)*sin(q2))^2 - Ixx3*(sin(q1)*sin(q2)*sin(q3) - cos(q2)*cos(q3)*sin(q1))^2 - Iyy3*(cos(q2)*sin(q1)*sin(q3) + cos(q3)*sin(q1)*sin(q2))^2 - Izz3*cos(q1)^2 + Izz3*sin(q1)^2)))/2 + 2*m3*(lc3*cos(q2)*sin(q1)*sin(q3) + lc3*cos(q3)*sin(q1)*sin(q2))*(l2*cos(q1)*sin(q2) + lc3*cos(q1)*cos(q2)*sin(q3) + lc3*cos(q1)*cos(q3)*sin(q2)));
     q3_d*((cos(q1)*(sin(q1)*(Ixx3*(cos(q1)*cos(q2)*cos(q3) - cos(q1)*sin(q2)*sin(q3))^2 + Iyy3*(cos(q1)*cos(q2)*sin(q3) + cos(q1)*cos(q3)*sin(q2))^2 + Izz3*sin(q1)^2) + cos(q1)*(Ixx3*(cos(q1)*cos(q2)*cos(q3) - cos(q1)*sin(q2)*sin(q3))*(sin(q1)*sin(q2)*sin(q3) - cos(q2)*cos(q3)*sin(q1)) - Iyy3*(cos(q1)*cos(q2)*sin(q3) + cos(q1)*cos(q3)*sin(q2))*(cos(q2)*sin(q1)*sin(q3) + cos(q3)*sin(q1)*sin(q2)) + Izz3*cos(q1)*sin(q1))))/2 + (sin(q1)*(cos(q1)*(Ixx3*(cos(q1)*cos(q2)*cos(q3) - cos(q1)*sin(q2)*sin(q3))^2 + Iyy3*(cos(q1)*cos(q2)*sin(q3) + cos(q1)*cos(q3)*sin(q2))^2 + Izz3*sin(q1)^2) - sin(q1)*(Ixx3*(cos(q1)*cos(q2)*cos(q3) - cos(q1)*sin(q2)*sin(q3))*(sin(q1)*sin(q2)*sin(q3) - cos(q2)*cos(q3)*sin(q1)) - Iyy3*(cos(q1)*cos(q2)*sin(q3) + cos(q1)*cos(q3)*sin(q2))*(cos(q2)*sin(q1)*sin(q3) + cos(q3)*sin(q1)*sin(q2)) + Izz3*cos(q1)*sin(q1)) + sin(q1)*(2*Ixx3*(cos(q1)*cos(q2)*cos(q3) - cos(q1)*sin(q2)*sin(q3))*(sin(q1)*sin(q2)*sin(q3) - cos(q2)*cos(q3)*sin(q1)) - 2*Iyy3*(cos(q1)*cos(q2)*sin(q3) + cos(q1)*cos(q3)*sin(q2))*(cos(q2)*sin(q1)*sin(q3) + cos(q3)*sin(q1)*sin(q2)) + 2*Izz3*cos(q1)*sin(q1)) - cos(q1)*(Ixx3*(cos(q1)*cos(q2)*cos(q3) - cos(q1)*sin(q2)*sin(q3))^2 + Iyy3*(cos(q1)*cos(q2)*sin(q3) + cos(q1)*cos(q3)*sin(q2))^2 - Ixx3*(sin(q1)*sin(q2)*sin(q3) - cos(q2)*cos(q3)*sin(q1))^2 - Iyy3*(cos(q2)*sin(q1)*sin(q3) + cos(q3)*sin(q1)*sin(q2))^2 - Izz3*cos(q1)^2 + Izz3*sin(q1)^2)))/2 - (sin(q1)*(cos(q1)*(Ixx3*(sin(q1)*sin(q2)*sin(q3) - cos(q2)*cos(q3)*sin(q1))^2 + Iyy3*(cos(q2)*sin(q1)*sin(q3) + cos(q3)*sin(q1)*sin(q2))^2 + Izz3*cos(q1)^2) + sin(q1)*(Ixx3*(cos(q1)*cos(q2)*cos(q3) - cos(q1)*sin(q2)*sin(q3))*(sin(q1)*sin(q2)*sin(q3) - cos(q2)*cos(q3)*sin(q1)) - Iyy3*(cos(q1)*cos(q2)*sin(q3) + cos(q1)*cos(q3)*sin(q2))*(cos(q2)*sin(q1)*sin(q3) + cos(q3)*sin(q1)*sin(q2)) + Izz3*cos(q1)*sin(q1))))/2 - (cos(q1)*(sin(q1)*(Ixx3*(sin(q1)*sin(q2)*sin(q3) - cos(q2)*cos(q3)*sin(q1))^2 + Iyy3*(cos(q2)*sin(q1)*sin(q3) + cos(q3)*sin(q1)*sin(q2))^2 + Izz3*cos(q1)^2) - cos(q1)*(Ixx3*(cos(q1)*cos(q2)*cos(q3) - cos(q1)*sin(q2)*sin(q3))*(sin(q1)*sin(q2)*sin(q3) - cos(q2)*cos(q3)*sin(q1)) - Iyy3*(cos(q1)*cos(q2)*sin(q3) + cos(q1)*cos(q3)*sin(q2))*(cos(q2)*sin(q1)*sin(q3) + cos(q3)*sin(q1)*sin(q2)) + Izz3*cos(q1)*sin(q1)) + cos(q1)*(2*Ixx3*(cos(q1)*cos(q2)*cos(q3) - cos(q1)*sin(q2)*sin(q3))*(sin(q1)*sin(q2)*sin(q3) - cos(q2)*cos(q3)*sin(q1)) - 2*Iyy3*(cos(q1)*cos(q2)*sin(q3) + cos(q1)*cos(q3)*sin(q2))*(cos(q2)*sin(q1)*sin(q3) + cos(q3)*sin(q1)*sin(q2)) + 2*Izz3*cos(q1)*sin(q1)) + sin(q1)*(Ixx3*(cos(q1)*cos(q2)*cos(q3) - cos(q1)*sin(q2)*sin(q3))^2 + Iyy3*(cos(q1)*cos(q2)*sin(q3) + cos(q1)*cos(q3)*sin(q2))^2 - Ixx3*(sin(q1)*sin(q2)*sin(q3) - cos(q2)*cos(q3)*sin(q1))^2 - Iyy3*(cos(q2)*sin(q1)*sin(q3) + cos(q3)*sin(q1)*sin(q2))^2 - Izz3*cos(q1)^2 + Izz3*sin(q1)^2)))/2 - sin(q1)*(Ixx3*(cos(q1)*cos(q2)*sin(q3) + cos(q1)*cos(q3)*sin(q2))*(cos(q2)*sin(q3) + cos(q3)*sin(q2)) - Ixx3*(cos(q1)*cos(q2)*cos(q3) - cos(q1)*sin(q2)*sin(q3))*(cos(q2)*cos(q3) - sin(q2)*sin(q3)) - Iyy3*(cos(q1)*cos(q2)*sin(q3) + cos(q1)*cos(q3)*sin(q2))*(cos(q2)*sin(q3) + cos(q3)*sin(q2)) + Iyy3*(cos(q1)*cos(q2)*cos(q3) - cos(q1)*sin(q2)*sin(q3))*(cos(q2)*cos(q3) - sin(q2)*sin(q3))) + cos(q1)*(Ixx3*(cos(q2)*sin(q1)*sin(q3) + cos(q3)*sin(q1)*sin(q2))*(cos(q2)*sin(q3) + cos(q3)*sin(q2)) + Ixx3*(sin(q1)*sin(q2)*sin(q3) - cos(q2)*cos(q3)*sin(q1))*(cos(q2)*cos(q3) - sin(q2)*sin(q3)) - Iyy3*(cos(q2)*sin(q1)*sin(q3) + cos(q3)*sin(q1)*sin(q2))*(cos(q2)*sin(q3) + cos(q3)*sin(q2)) - Iyy3*(sin(q1)*sin(q2)*sin(q3) - cos(q2)*cos(q3)*sin(q1))*(cos(q2)*cos(q3) - sin(q2)*sin(q3))) - 4*m3*(lc3*cos(q1)*cos(q2)*sin(q3) + lc3*cos(q1)*cos(q3)*sin(q2))*(lc3*cos(q2)*sin(q1)*sin(q3) + lc3*cos(q3)*sin(q1)*sin(q2)) + 2*m3*(lc3*cos(q1)*cos(q2)*cos(q3) - lc3*cos(q1)*sin(q2)*sin(q3))*(l2*cos(q2)*sin(q1) + lc3*cos(q2)*cos(q3)*sin(q1) - lc3*sin(q1)*sin(q2)*sin(q3))) - q2_d*((sin(q1)*(cos(q1)*(Ixx3*(sin(q1)*sin(q2)*sin(q3) - cos(q2)*cos(q3)*sin(q1))^2 + Iyy3*(cos(q2)*sin(q1)*sin(q3) + cos(q3)*sin(q1)*sin(q2))^2 + Izz3*cos(q1)^2) + sin(q1)*(Ixx3*(cos(q1)*cos(q2)*cos(q3) - cos(q1)*sin(q2)*sin(q3))*(sin(q1)*sin(q2)*sin(q3) - cos(q2)*cos(q3)*sin(q1)) - Iyy3*(cos(q1)*cos(q2)*sin(q3) + cos(q1)*cos(q3)*sin(q2))*(cos(q2)*sin(q1)*sin(q3) + cos(q3)*sin(q1)*sin(q2)) + Izz3*cos(q1)*sin(q1))))/2 - (sin(q1)*(cos(q1)*(Ixx3*(cos(q1)*cos(q2)*cos(q3) - cos(q1)*sin(q2)*sin(q3))^2 + Iyy3*(cos(q1)*cos(q2)*sin(q3) + cos(q1)*cos(q3)*sin(q2))^2 + Izz3*sin(q1)^2) - sin(q1)*(Ixx3*(cos(q1)*cos(q2)*cos(q3) - cos(q1)*sin(q2)*sin(q3))*(sin(q1)*sin(q2)*sin(q3) - cos(q2)*cos(q3)*sin(q1)) - Iyy3*(cos(q1)*cos(q2)*sin(q3) + cos(q1)*cos(q3)*sin(q2))*(cos(q2)*sin(q1)*sin(q3) + cos(q3)*sin(q1)*sin(q2)) + Izz3*cos(q1)*sin(q1)) + sin(q1)*(2*Ixx3*(cos(q1)*cos(q2)*cos(q3) - cos(q1)*sin(q2)*sin(q3))*(sin(q1)*sin(q2)*sin(q3) - cos(q2)*cos(q3)*sin(q1)) - 2*Iyy3*(cos(q1)*cos(q2)*sin(q3) + cos(q1)*cos(q3)*sin(q2))*(cos(q2)*sin(q1)*sin(q3) + cos(q3)*sin(q1)*sin(q2)) + 2*Izz3*cos(q1)*sin(q1)) - cos(q1)*(Ixx3*(cos(q1)*cos(q2)*cos(q3) - cos(q1)*sin(q2)*sin(q3))^2 + Iyy3*(cos(q1)*cos(q2)*sin(q3) + cos(q1)*cos(q3)*sin(q2))^2 - Ixx3*(sin(q1)*sin(q2)*sin(q3) - cos(q2)*cos(q3)*sin(q1))^2 - Iyy3*(cos(q2)*sin(q1)*sin(q3) + cos(q3)*sin(q1)*sin(q2))^2 - Izz3*cos(q1)^2 + Izz3*sin(q1)^2)))/2 - (cos(q1)*(sin(q1)*(Ixx3*(cos(q1)*cos(q2)*cos(q3) - cos(q1)*sin(q2)*sin(q3))^2 + Iyy3*(cos(q1)*cos(q2)*sin(q3) + cos(q1)*cos(q3)*sin(q2))^2 + Izz3*sin(q1)^2) + cos(q1)*(Ixx3*(cos(q1)*cos(q2)*cos(q3) - cos(q1)*sin(q2)*sin(q3))*(sin(q1)*sin(q2)*sin(q3) - cos(q2)*cos(q3)*sin(q1)) - Iyy3*(cos(q1)*cos(q2)*sin(q3) + cos(q1)*cos(q3)*sin(q2))*(cos(q2)*sin(q1)*sin(q3) + cos(q3)*sin(q1)*sin(q2)) + Izz3*cos(q1)*sin(q1))))/2 + (cos(q1)*(sin(q1)*(Ixx3*(sin(q1)*sin(q2)*sin(q3) - cos(q2)*cos(q3)*sin(q1))^2 + Iyy3*(cos(q2)*sin(q1)*sin(q3) + cos(q3)*sin(q1)*sin(q2))^2 + Izz3*cos(q1)^2) - cos(q1)*(Ixx3*(cos(q1)*cos(q2)*cos(q3) - cos(q1)*sin(q2)*sin(q3))*(sin(q1)*sin(q2)*sin(q3) - cos(q2)*cos(q3)*sin(q1)) - Iyy3*(cos(q1)*cos(q2)*sin(q3) + cos(q1)*cos(q3)*sin(q2))*(cos(q2)*sin(q1)*sin(q3) + cos(q3)*sin(q1)*sin(q2)) + Izz3*cos(q1)*sin(q1)) + cos(q1)*(2*Ixx3*(cos(q1)*cos(q2)*cos(q3) - cos(q1)*sin(q2)*sin(q3))*(sin(q1)*sin(q2)*sin(q3) - cos(q2)*cos(q3)*sin(q1)) - 2*Iyy3*(cos(q1)*cos(q2)*sin(q3) + cos(q1)*cos(q3)*sin(q2))*(cos(q2)*sin(q1)*sin(q3) + cos(q3)*sin(q1)*sin(q2)) + 2*Izz3*cos(q1)*sin(q1)) + sin(q1)*(Ixx3*(cos(q1)*cos(q2)*cos(q3) - cos(q1)*sin(q2)*sin(q3))^2 + Iyy3*(cos(q1)*cos(q2)*sin(q3) + cos(q1)*cos(q3)*sin(q2))^2 - Ixx3*(sin(q1)*sin(q2)*sin(q3) - cos(q2)*cos(q3)*sin(q1))^2 - Iyy3*(cos(q2)*sin(q1)*sin(q3) + cos(q3)*sin(q1)*sin(q2))^2 - Izz3*cos(q1)^2 + Izz3*sin(q1)^2)))/2 + sin(q1)*(Ixx3*(cos(q1)*cos(q2)*sin(q3) + cos(q1)*cos(q3)*sin(q2))*(cos(q2)*sin(q3) + cos(q3)*sin(q2)) - Ixx3*(cos(q1)*cos(q2)*cos(q3) - cos(q1)*sin(q2)*sin(q3))*(cos(q2)*cos(q3) - sin(q2)*sin(q3)) - Iyy3*(cos(q1)*cos(q2)*sin(q3) + cos(q1)*cos(q3)*sin(q2))*(cos(q2)*sin(q3) + cos(q3)*sin(q2)) + Iyy3*(cos(q1)*cos(q2)*cos(q3) - cos(q1)*sin(q2)*sin(q3))*(cos(q2)*cos(q3) - sin(q2)*sin(q3))) - cos(q1)*(Ixx3*(cos(q2)*sin(q1)*sin(q3) + cos(q3)*sin(q1)*sin(q2))*(cos(q2)*sin(q3) + cos(q3)*sin(q2)) + Ixx3*(sin(q1)*sin(q2)*sin(q3) - cos(q2)*cos(q3)*sin(q1))*(cos(q2)*cos(q3) - sin(q2)*sin(q3)) - Iyy3*(cos(q2)*sin(q1)*sin(q3) + cos(q3)*sin(q1)*sin(q2))*(cos(q2)*sin(q3) + cos(q3)*sin(q2)) - Iyy3*(sin(q1)*sin(q2)*sin(q3) - cos(q2)*cos(q3)*sin(q1))*(cos(q2)*cos(q3) - sin(q2)*sin(q3))) + 2*m3*(lc3*cos(q2)*sin(q1)*sin(q3) + lc3*cos(q3)*sin(q1)*sin(q2))*(l2*cos(q1)*sin(q2) + lc3*cos(q1)*cos(q2)*sin(q3) + lc3*cos(q1)*cos(q3)*sin(q2)) - 2*m3*(lc3*cos(q1)*cos(q2)*cos(q3) - lc3*cos(q1)*sin(q2)*sin(q3))*(l2*cos(q2)*sin(q1) + lc3*cos(q2)*cos(q3)*sin(q1) - lc3*sin(q1)*sin(q2)*sin(q3)) + 2*m3*(lc3*cos(q1)*cos(q2)*sin(q3) + lc3*cos(q1)*cos(q3)*sin(q2))*(l2*sin(q1)*sin(q2) + lc3*cos(q2)*sin(q1)*sin(q3) + lc3*cos(q3)*sin(q1)*sin(q2))) + q1_d*(2*m3*(lc3*cos(q1)*cos(q2)*sin(q3) + lc3*cos(q1)*cos(q3)*sin(q2))*(l2*cos(q1)*cos(q2) + lc3*cos(q1)*cos(q2)*cos(q3) - lc3*cos(q1)*sin(q2)*sin(q3)) - 4*m3*(lc3*cos(q2)*sin(q1)*sin(q3) + lc3*cos(q3)*sin(q1)*sin(q2))*(l2*cos(q2)*sin(q1) + lc3*cos(q2)*cos(q3)*sin(q1) - lc3*sin(q1)*sin(q2)*sin(q3)) + Ixx3*(cos(q2)*sin(q3) + cos(q3)*sin(q2))*(cos(q2)*cos(q3) - sin(q2)*sin(q3)) - Iyy3*(cos(q2)*sin(q3) + cos(q3)*sin(q2))*(cos(q2)*cos(q3) - sin(q2)*sin(q3))), q2_d*((3*cos(q1)*(cos(q1)*(2*Ixx3*(cos(q2)*sin(q1)*sin(q3) + cos(q3)*sin(q1)*sin(q2))*(sin(q1)*sin(q2)*sin(q3) - cos(q2)*cos(q3)*sin(q1)) - 2*Iyy3*(cos(q2)*sin(q1)*sin(q3) + cos(q3)*sin(q1)*sin(q2))*(sin(q1)*sin(q2)*sin(q3) - cos(q2)*cos(q3)*sin(q1))) - sin(q1)*(Ixx3*(cos(q1)*cos(q2)*sin(q3) + cos(q1)*cos(q3)*sin(q2))*(sin(q1)*sin(q2)*sin(q3) - cos(q2)*cos(q3)*sin(q1)) - Ixx3*(cos(q1)*cos(q2)*cos(q3) - cos(q1)*sin(q2)*sin(q3))*(cos(q2)*sin(q1)*sin(q3) + cos(q3)*sin(q1)*sin(q2)) - Iyy3*(cos(q1)*cos(q2)*sin(q3) + cos(q1)*cos(q3)*sin(q2))*(sin(q1)*sin(q2)*sin(q3) - cos(q2)*cos(q3)*sin(q1)) + Iyy3*(cos(q1)*cos(q2)*cos(q3) - cos(q1)*sin(q2)*sin(q3))*(cos(q2)*sin(q1)*sin(q3) + cos(q3)*sin(q1)*sin(q2)))))/2 - (3*sin(q1)*(cos(q1)*(Ixx3*(cos(q1)*cos(q2)*sin(q3) + cos(q1)*cos(q3)*sin(q2))*(sin(q1)*sin(q2)*sin(q3) - cos(q2)*cos(q3)*sin(q1)) - Ixx3*(cos(q1)*cos(q2)*cos(q3) - cos(q1)*sin(q2)*sin(q3))*(cos(q2)*sin(q1)*sin(q3) + cos(q3)*sin(q1)*sin(q2)) - Iyy3*(cos(q1)*cos(q2)*sin(q3) + cos(q1)*cos(q3)*sin(q2))*(sin(q1)*sin(q2)*sin(q3) - cos(q2)*cos(q3)*sin(q1)) + Iyy3*(cos(q1)*cos(q2)*cos(q3) - cos(q1)*sin(q2)*sin(q3))*(cos(q2)*sin(q1)*sin(q3) + cos(q3)*sin(q1)*sin(q2))) + sin(q1)*(2*Ixx3*(cos(q1)*cos(q2)*sin(q3) + cos(q1)*cos(q3)*sin(q2))*(cos(q1)*cos(q2)*cos(q3) - cos(q1)*sin(q2)*sin(q3)) - 2*Iyy3*(cos(q1)*cos(q2)*sin(q3) + cos(q1)*cos(q3)*sin(q2))*(cos(q1)*cos(q2)*cos(q3) - cos(q1)*sin(q2)*sin(q3)))))/2 - 2*m3*(lc3*cos(q2)*sin(q3) + lc3*cos(q3)*sin(q2))*(cos(q2)*(l1 + l2) + lc3*cos(q2)*cos(q3) - lc3*sin(q2)*sin(q3)) - m3*(lc3*cos(q2)*cos(q3) - lc3*sin(q2)*sin(q3))*(sin(q2)*(l1 + l2) + lc3*cos(q2)*sin(q3) + lc3*cos(q3)*sin(q2)) + 2*m3*(lc3*cos(q1)*cos(q2)*sin(q3) + lc3*cos(q1)*cos(q3)*sin(q2))*(l2*cos(q1)*cos(q2) + lc3*cos(q1)*cos(q2)*cos(q3) - lc3*cos(q1)*sin(q2)*sin(q3)) + 4*m3*(lc3*cos(q1)*cos(q2)*cos(q3) - lc3*cos(q1)*sin(q2)*sin(q3))*(l2*cos(q1)*sin(q2) + lc3*cos(q1)*cos(q2)*sin(q3) + lc3*cos(q1)*cos(q3)*sin(q2))) - q1_d*((sin(q1)*(cos(q1)*(Ixx3*(sin(q1)*sin(q2)*sin(q3) - cos(q2)*cos(q3)*sin(q1))^2 + Iyy3*(cos(q2)*sin(q1)*sin(q3) + cos(q3)*sin(q1)*sin(q2))^2 + Izz3*cos(q1)^2) + sin(q1)*(Ixx3*(cos(q1)*cos(q2)*cos(q3) - cos(q1)*sin(q2)*sin(q3))*(sin(q1)*sin(q2)*sin(q3) - cos(q2)*cos(q3)*sin(q1)) - Iyy3*(cos(q1)*cos(q2)*sin(q3) + cos(q1)*cos(q3)*sin(q2))*(cos(q2)*sin(q1)*sin(q3) + cos(q3)*sin(q1)*sin(q2)) + Izz3*cos(q1)*sin(q1))))/2 - (sin(q1)*(cos(q1)*(Ixx3*(cos(q1)*cos(q2)*cos(q3) - cos(q1)*sin(q2)*sin(q3))^2 + Iyy3*(cos(q1)*cos(q2)*sin(q3) + cos(q1)*cos(q3)*sin(q2))^2 + Izz3*sin(q1)^2) - sin(q1)*(Ixx3*(cos(q1)*cos(q2)*cos(q3) - cos(q1)*sin(q2)*sin(q3))*(sin(q1)*sin(q2)*sin(q3) - cos(q2)*cos(q3)*sin(q1)) - Iyy3*(cos(q1)*cos(q2)*sin(q3) + cos(q1)*cos(q3)*sin(q2))*(cos(q2)*sin(q1)*sin(q3) + cos(q3)*sin(q1)*sin(q2)) + Izz3*cos(q1)*sin(q1)) + sin(q1)*(2*Ixx3*(cos(q1)*cos(q2)*cos(q3) - cos(q1)*sin(q2)*sin(q3))*(sin(q1)*sin(q2)*sin(q3) - cos(q2)*cos(q3)*sin(q1)) - 2*Iyy3*(cos(q1)*cos(q2)*sin(q3) + cos(q1)*cos(q3)*sin(q2))*(cos(q2)*sin(q1)*sin(q3) + cos(q3)*sin(q1)*sin(q2)) + 2*Izz3*cos(q1)*sin(q1)) - cos(q1)*(Ixx3*(cos(q1)*cos(q2)*cos(q3) - cos(q1)*sin(q2)*sin(q3))^2 + Iyy3*(cos(q1)*cos(q2)*sin(q3) + cos(q1)*cos(q3)*sin(q2))^2 - Ixx3*(sin(q1)*sin(q2)*sin(q3) - cos(q2)*cos(q3)*sin(q1))^2 - Iyy3*(cos(q2)*sin(q1)*sin(q3) + cos(q3)*sin(q1)*sin(q2))^2 - Izz3*cos(q1)^2 + Izz3*sin(q1)^2)))/2 - (cos(q1)*(sin(q1)*(Ixx3*(cos(q1)*cos(q2)*cos(q3) - cos(q1)*sin(q2)*sin(q3))^2 + Iyy3*(cos(q1)*cos(q2)*sin(q3) + cos(q1)*cos(q3)*sin(q2))^2 + Izz3*sin(q1)^2) + cos(q1)*(Ixx3*(cos(q1)*cos(q2)*cos(q3) - cos(q1)*sin(q2)*sin(q3))*(sin(q1)*sin(q2)*sin(q3) - cos(q2)*cos(q3)*sin(q1)) - Iyy3*(cos(q1)*cos(q2)*sin(q3) + cos(q1)*cos(q3)*sin(q2))*(cos(q2)*sin(q1)*sin(q3) + cos(q3)*sin(q1)*sin(q2)) + Izz3*cos(q1)*sin(q1))))/2 + (cos(q1)*(sin(q1)*(Ixx3*(sin(q1)*sin(q2)*sin(q3) - cos(q2)*cos(q3)*sin(q1))^2 + Iyy3*(cos(q2)*sin(q1)*sin(q3) + cos(q3)*sin(q1)*sin(q2))^2 + Izz3*cos(q1)^2) - cos(q1)*(Ixx3*(cos(q1)*cos(q2)*cos(q3) - cos(q1)*sin(q2)*sin(q3))*(sin(q1)*sin(q2)*sin(q3) - cos(q2)*cos(q3)*sin(q1)) - Iyy3*(cos(q1)*cos(q2)*sin(q3) + cos(q1)*cos(q3)*sin(q2))*(cos(q2)*sin(q1)*sin(q3) + cos(q3)*sin(q1)*sin(q2)) + Izz3*cos(q1)*sin(q1)) + cos(q1)*(2*Ixx3*(cos(q1)*cos(q2)*cos(q3) - cos(q1)*sin(q2)*sin(q3))*(sin(q1)*sin(q2)*sin(q3) - cos(q2)*cos(q3)*sin(q1)) - 2*Iyy3*(cos(q1)*cos(q2)*sin(q3) + cos(q1)*cos(q3)*sin(q2))*(cos(q2)*sin(q1)*sin(q3) + cos(q3)*sin(q1)*sin(q2)) + 2*Izz3*cos(q1)*sin(q1)) + sin(q1)*(Ixx3*(cos(q1)*cos(q2)*cos(q3) - cos(q1)*sin(q2)*sin(q3))^2 + Iyy3*(cos(q1)*cos(q2)*sin(q3) + cos(q1)*cos(q3)*sin(q2))^2 - Ixx3*(sin(q1)*sin(q2)*sin(q3) - cos(q2)*cos(q3)*sin(q1))^2 - Iyy3*(cos(q2)*sin(q1)*sin(q3) + cos(q3)*sin(q1)*sin(q2))^2 - Izz3*cos(q1)^2 + Izz3*sin(q1)^2)))/2 + sin(q1)*(Ixx3*(cos(q1)*cos(q2)*sin(q3) + cos(q1)*cos(q3)*sin(q2))*(cos(q2)*sin(q3) + cos(q3)*sin(q2)) - Ixx3*(cos(q1)*cos(q2)*cos(q3) - cos(q1)*sin(q2)*sin(q3))*(cos(q2)*cos(q3) - sin(q2)*sin(q3)) - Iyy3*(cos(q1)*cos(q2)*sin(q3) + cos(q1)*cos(q3)*sin(q2))*(cos(q2)*sin(q3) + cos(q3)*sin(q2)) + Iyy3*(cos(q1)*cos(q2)*cos(q3) - cos(q1)*sin(q2)*sin(q3))*(cos(q2)*cos(q3) - sin(q2)*sin(q3))) - cos(q1)*(Ixx3*(cos(q2)*sin(q1)*sin(q3) + cos(q3)*sin(q1)*sin(q2))*(cos(q2)*sin(q3) + cos(q3)*sin(q2)) + Ixx3*(sin(q1)*sin(q2)*sin(q3) - cos(q2)*cos(q3)*sin(q1))*(cos(q2)*cos(q3) - sin(q2)*sin(q3)) - Iyy3*(cos(q2)*sin(q1)*sin(q3) + cos(q3)*sin(q1)*sin(q2))*(cos(q2)*sin(q3) + cos(q3)*sin(q2)) - Iyy3*(sin(q1)*sin(q2)*sin(q3) - cos(q2)*cos(q3)*sin(q1))*(cos(q2)*cos(q3) - sin(q2)*sin(q3))) + 2*m3*(lc3*cos(q2)*sin(q1)*sin(q3) + lc3*cos(q3)*sin(q1)*sin(q2))*(l2*cos(q1)*sin(q2) + lc3*cos(q1)*cos(q2)*sin(q3) + lc3*cos(q1)*cos(q3)*sin(q2)) - 2*m3*(lc3*cos(q1)*cos(q2)*cos(q3) - lc3*cos(q1)*sin(q2)*sin(q3))*(l2*cos(q2)*sin(q1) + lc3*cos(q2)*cos(q3)*sin(q1) - lc3*sin(q1)*sin(q2)*sin(q3)) + 2*m3*(lc3*cos(q1)*cos(q2)*sin(q3) + lc3*cos(q1)*cos(q3)*sin(q2))*(l2*sin(q1)*sin(q2) + lc3*cos(q2)*sin(q1)*sin(q3) + lc3*cos(q3)*sin(q1)*sin(q2))) + q3_d*((3*cos(q1)*(cos(q1)*(2*Ixx3*(cos(q2)*sin(q1)*sin(q3) + cos(q3)*sin(q1)*sin(q2))*(sin(q1)*sin(q2)*sin(q3) - cos(q2)*cos(q3)*sin(q1)) - 2*Iyy3*(cos(q2)*sin(q1)*sin(q3) + cos(q3)*sin(q1)*sin(q2))*(sin(q1)*sin(q2)*sin(q3) - cos(q2)*cos(q3)*sin(q1))) - sin(q1)*(Ixx3*(cos(q1)*cos(q2)*sin(q3) + cos(q1)*cos(q3)*sin(q2))*(sin(q1)*sin(q2)*sin(q3) - cos(q2)*cos(q3)*sin(q1)) - Ixx3*(cos(q1)*cos(q2)*cos(q3) - cos(q1)*sin(q2)*sin(q3))*(cos(q2)*sin(q1)*sin(q3) + cos(q3)*sin(q1)*sin(q2)) - Iyy3*(cos(q1)*cos(q2)*sin(q3) + cos(q1)*cos(q3)*sin(q2))*(sin(q1)*sin(q2)*sin(q3) - cos(q2)*cos(q3)*sin(q1)) + Iyy3*(cos(q1)*cos(q2)*cos(q3) - cos(q1)*sin(q2)*sin(q3))*(cos(q2)*sin(q1)*sin(q3) + cos(q3)*sin(q1)*sin(q2)))))/2 - (3*sin(q1)*(cos(q1)*(Ixx3*(cos(q1)*cos(q2)*sin(q3) + cos(q1)*cos(q3)*sin(q2))*(sin(q1)*sin(q2)*sin(q3) - cos(q2)*cos(q3)*sin(q1)) - Ixx3*(cos(q1)*cos(q2)*cos(q3) - cos(q1)*sin(q2)*sin(q3))*(cos(q2)*sin(q1)*sin(q3) + cos(q3)*sin(q1)*sin(q2)) - Iyy3*(cos(q1)*cos(q2)*sin(q3) + cos(q1)*cos(q3)*sin(q2))*(sin(q1)*sin(q2)*sin(q3) - cos(q2)*cos(q3)*sin(q1)) + Iyy3*(cos(q1)*cos(q2)*cos(q3) - cos(q1)*sin(q2)*sin(q3))*(cos(q2)*sin(q1)*sin(q3) + cos(q3)*sin(q1)*sin(q2))) + sin(q1)*(2*Ixx3*(cos(q1)*cos(q2)*sin(q3) + cos(q1)*cos(q3)*sin(q2))*(cos(q1)*cos(q2)*cos(q3) - cos(q1)*sin(q2)*sin(q3)) - 2*Iyy3*(cos(q1)*cos(q2)*sin(q3) + cos(q1)*cos(q3)*sin(q2))*(cos(q1)*cos(q2)*cos(q3) - cos(q1)*sin(q2)*sin(q3)))))/2 - m3*(lc3*cos(q2)*sin(q3) + lc3*cos(q3)*sin(q2))*(cos(q2)*(l1 + l2) + lc3*cos(q2)*cos(q3) - lc3*sin(q2)*sin(q3)) + 2*m3*(lc3*cos(q1)*cos(q2)*cos(q3) - lc3*cos(q1)*sin(q2)*sin(q3))*(l2*cos(q1)*sin(q2) + lc3*cos(q1)*cos(q2)*sin(q3) + lc3*cos(q1)*cos(q3)*sin(q2)) - 2*m3*(lc3*cos(q2)*sin(q3) + lc3*cos(q3)*sin(q2))*(lc3*cos(q2)*cos(q3) - lc3*sin(q2)*sin(q3)) + 4*m3*(lc3*cos(q1)*cos(q2)*sin(q3) + lc3*cos(q1)*cos(q3)*sin(q2))*(lc3*cos(q1)*cos(q2)*cos(q3) - lc3*cos(q1)*sin(q2)*sin(q3))), q1_d*((cos(q1)*(sin(q1)*(Ixx3*(cos(q1)*cos(q2)*cos(q3) - cos(q1)*sin(q2)*sin(q3))^2 + Iyy3*(cos(q1)*cos(q2)*sin(q3) + cos(q1)*cos(q3)*sin(q2))^2 + Izz3*sin(q1)^2) + cos(q1)*(Ixx3*(cos(q1)*cos(q2)*cos(q3) - cos(q1)*sin(q2)*sin(q3))*(sin(q1)*sin(q2)*sin(q3) - cos(q2)*cos(q3)*sin(q1)) - Iyy3*(cos(q1)*cos(q2)*sin(q3) + cos(q1)*cos(q3)*sin(q2))*(cos(q2)*sin(q1)*sin(q3) + cos(q3)*sin(q1)*sin(q2)) + Izz3*cos(q1)*sin(q1))))/2 + (sin(q1)*(cos(q1)*(Ixx3*(cos(q1)*cos(q2)*cos(q3) - cos(q1)*sin(q2)*sin(q3))^2 + Iyy3*(cos(q1)*cos(q2)*sin(q3) + cos(q1)*cos(q3)*sin(q2))^2 + Izz3*sin(q1)^2) - sin(q1)*(Ixx3*(cos(q1)*cos(q2)*cos(q3) - cos(q1)*sin(q2)*sin(q3))*(sin(q1)*sin(q2)*sin(q3) - cos(q2)*cos(q3)*sin(q1)) - Iyy3*(cos(q1)*cos(q2)*sin(q3) + cos(q1)*cos(q3)*sin(q2))*(cos(q2)*sin(q1)*sin(q3) + cos(q3)*sin(q1)*sin(q2)) + Izz3*cos(q1)*sin(q1)) + sin(q1)*(2*Ixx3*(cos(q1)*cos(q2)*cos(q3) - cos(q1)*sin(q2)*sin(q3))*(sin(q1)*sin(q2)*sin(q3) - cos(q2)*cos(q3)*sin(q1)) - 2*Iyy3*(cos(q1)*cos(q2)*sin(q3) + cos(q1)*cos(q3)*sin(q2))*(cos(q2)*sin(q1)*sin(q3) + cos(q3)*sin(q1)*sin(q2)) + 2*Izz3*cos(q1)*sin(q1)) - cos(q1)*(Ixx3*(cos(q1)*cos(q2)*cos(q3) - cos(q1)*sin(q2)*sin(q3))^2 + Iyy3*(cos(q1)*cos(q2)*sin(q3) + cos(q1)*cos(q3)*sin(q2))^2 - Ixx3*(sin(q1)*sin(q2)*sin(q3) - cos(q2)*cos(q3)*sin(q1))^2 - Iyy3*(cos(q2)*sin(q1)*sin(q3) + cos(q3)*sin(q1)*sin(q2))^2 - Izz3*cos(q1)^2 + Izz3*sin(q1)^2)))/2 - (sin(q1)*(cos(q1)*(Ixx3*(sin(q1)*sin(q2)*sin(q3) - cos(q2)*cos(q3)*sin(q1))^2 + Iyy3*(cos(q2)*sin(q1)*sin(q3) + cos(q3)*sin(q1)*sin(q2))^2 + Izz3*cos(q1)^2) + sin(q1)*(Ixx3*(cos(q1)*cos(q2)*cos(q3) - cos(q1)*sin(q2)*sin(q3))*(sin(q1)*sin(q2)*sin(q3) - cos(q2)*cos(q3)*sin(q1)) - Iyy3*(cos(q1)*cos(q2)*sin(q3) + cos(q1)*cos(q3)*sin(q2))*(cos(q2)*sin(q1)*sin(q3) + cos(q3)*sin(q1)*sin(q2)) + Izz3*cos(q1)*sin(q1))))/2 - (cos(q1)*(sin(q1)*(Ixx3*(sin(q1)*sin(q2)*sin(q3) - cos(q2)*cos(q3)*sin(q1))^2 + Iyy3*(cos(q2)*sin(q1)*sin(q3) + cos(q3)*sin(q1)*sin(q2))^2 + Izz3*cos(q1)^2) - cos(q1)*(Ixx3*(cos(q1)*cos(q2)*cos(q3) - cos(q1)*sin(q2)*sin(q3))*(sin(q1)*sin(q2)*sin(q3) - cos(q2)*cos(q3)*sin(q1)) - Iyy3*(cos(q1)*cos(q2)*sin(q3) + cos(q1)*cos(q3)*sin(q2))*(cos(q2)*sin(q1)*sin(q3) + cos(q3)*sin(q1)*sin(q2)) + Izz3*cos(q1)*sin(q1)) + cos(q1)*(2*Ixx3*(cos(q1)*cos(q2)*cos(q3) - cos(q1)*sin(q2)*sin(q3))*(sin(q1)*sin(q2)*sin(q3) - cos(q2)*cos(q3)*sin(q1)) - 2*Iyy3*(cos(q1)*cos(q2)*sin(q3) + cos(q1)*cos(q3)*sin(q2))*(cos(q2)*sin(q1)*sin(q3) + cos(q3)*sin(q1)*sin(q2)) + 2*Izz3*cos(q1)*sin(q1)) + sin(q1)*(Ixx3*(cos(q1)*cos(q2)*cos(q3) - cos(q1)*sin(q2)*sin(q3))^2 + Iyy3*(cos(q1)*cos(q2)*sin(q3) + cos(q1)*cos(q3)*sin(q2))^2 - Ixx3*(sin(q1)*sin(q2)*sin(q3) - cos(q2)*cos(q3)*sin(q1))^2 - Iyy3*(cos(q2)*sin(q1)*sin(q3) + cos(q3)*sin(q1)*sin(q2))^2 - Izz3*cos(q1)^2 + Izz3*sin(q1)^2)))/2 - sin(q1)*(Ixx3*(cos(q1)*cos(q2)*sin(q3) + cos(q1)*cos(q3)*sin(q2))*(cos(q2)*sin(q3) + cos(q3)*sin(q2)) - Ixx3*(cos(q1)*cos(q2)*cos(q3) - cos(q1)*sin(q2)*sin(q3))*(cos(q2)*cos(q3) - sin(q2)*sin(q3)) - Iyy3*(cos(q1)*cos(q2)*sin(q3) + cos(q1)*cos(q3)*sin(q2))*(cos(q2)*sin(q3) + cos(q3)*sin(q2)) + Iyy3*(cos(q1)*cos(q2)*cos(q3) - cos(q1)*sin(q2)*sin(q3))*(cos(q2)*cos(q3) - sin(q2)*sin(q3))) + cos(q1)*(Ixx3*(cos(q2)*sin(q1)*sin(q3) + cos(q3)*sin(q1)*sin(q2))*(cos(q2)*sin(q3) + cos(q3)*sin(q2)) + Ixx3*(sin(q1)*sin(q2)*sin(q3) - cos(q2)*cos(q3)*sin(q1))*(cos(q2)*cos(q3) - sin(q2)*sin(q3)) - Iyy3*(cos(q2)*sin(q1)*sin(q3) + cos(q3)*sin(q1)*sin(q2))*(cos(q2)*sin(q3) + cos(q3)*sin(q2)) - Iyy3*(sin(q1)*sin(q2)*sin(q3) - cos(q2)*cos(q3)*sin(q1))*(cos(q2)*cos(q3) - sin(q2)*sin(q3))) - 4*m3*(lc3*cos(q1)*cos(q2)*sin(q3) + lc3*cos(q1)*cos(q3)*sin(q2))*(lc3*cos(q2)*sin(q1)*sin(q3) + lc3*cos(q3)*sin(q1)*sin(q2)) + 2*m3*(lc3*cos(q1)*cos(q2)*cos(q3) - lc3*cos(q1)*sin(q2)*sin(q3))*(l2*cos(q2)*sin(q1) + lc3*cos(q2)*cos(q3)*sin(q1) - lc3*sin(q1)*sin(q2)*sin(q3))) + q3_d*((3*cos(q1)*(cos(q1)*(2*Ixx3*(cos(q2)*sin(q1)*sin(q3) + cos(q3)*sin(q1)*sin(q2))*(sin(q1)*sin(q2)*sin(q3) - cos(q2)*cos(q3)*sin(q1)) - 2*Iyy3*(cos(q2)*sin(q1)*sin(q3) + cos(q3)*sin(q1)*sin(q2))*(sin(q1)*sin(q2)*sin(q3) - cos(q2)*cos(q3)*sin(q1))) - sin(q1)*(Ixx3*(cos(q1)*cos(q2)*sin(q3) + cos(q1)*cos(q3)*sin(q2))*(sin(q1)*sin(q2)*sin(q3) - cos(q2)*cos(q3)*sin(q1)) - Ixx3*(cos(q1)*cos(q2)*cos(q3) - cos(q1)*sin(q2)*sin(q3))*(cos(q2)*sin(q1)*sin(q3) + cos(q3)*sin(q1)*sin(q2)) - Iyy3*(cos(q1)*cos(q2)*sin(q3) + cos(q1)*cos(q3)*sin(q2))*(sin(q1)*sin(q2)*sin(q3) - cos(q2)*cos(q3)*sin(q1)) + Iyy3*(cos(q1)*cos(q2)*cos(q3) - cos(q1)*sin(q2)*sin(q3))*(cos(q2)*sin(q1)*sin(q3) + cos(q3)*sin(q1)*sin(q2)))))/2 - (3*sin(q1)*(cos(q1)*(Ixx3*(cos(q1)*cos(q2)*sin(q3) + cos(q1)*cos(q3)*sin(q2))*(sin(q1)*sin(q2)*sin(q3) - cos(q2)*cos(q3)*sin(q1)) - Ixx3*(cos(q1)*cos(q2)*cos(q3) - cos(q1)*sin(q2)*sin(q3))*(cos(q2)*sin(q1)*sin(q3) + cos(q3)*sin(q1)*sin(q2)) - Iyy3*(cos(q1)*cos(q2)*sin(q3) + cos(q1)*cos(q3)*sin(q2))*(sin(q1)*sin(q2)*sin(q3) - cos(q2)*cos(q3)*sin(q1)) + Iyy3*(cos(q1)*cos(q2)*cos(q3) - cos(q1)*sin(q2)*sin(q3))*(cos(q2)*sin(q1)*sin(q3) + cos(q3)*sin(q1)*sin(q2))) + sin(q1)*(2*Ixx3*(cos(q1)*cos(q2)*sin(q3) + cos(q1)*cos(q3)*sin(q2))*(cos(q1)*cos(q2)*cos(q3) - cos(q1)*sin(q2)*sin(q3)) - 2*Iyy3*(cos(q1)*cos(q2)*sin(q3) + cos(q1)*cos(q3)*sin(q2))*(cos(q1)*cos(q2)*cos(q3) - cos(q1)*sin(q2)*sin(q3)))))/2 - 3*m3*(lc3*cos(q2)*sin(q3) + lc3*cos(q3)*sin(q2))*(lc3*cos(q2)*cos(q3) - lc3*sin(q2)*sin(q3)) + 6*m3*(lc3*cos(q1)*cos(q2)*sin(q3) + lc3*cos(q1)*cos(q3)*sin(q2))*(lc3*cos(q1)*cos(q2)*cos(q3) - lc3*cos(q1)*sin(q2)*sin(q3))) + q2_d*((3*cos(q1)*(cos(q1)*(2*Ixx3*(cos(q2)*sin(q1)*sin(q3) + cos(q3)*sin(q1)*sin(q2))*(sin(q1)*sin(q2)*sin(q3) - cos(q2)*cos(q3)*sin(q1)) - 2*Iyy3*(cos(q2)*sin(q1)*sin(q3) + cos(q3)*sin(q1)*sin(q2))*(sin(q1)*sin(q2)*sin(q3) - cos(q2)*cos(q3)*sin(q1))) - sin(q1)*(Ixx3*(cos(q1)*cos(q2)*sin(q3) + cos(q1)*cos(q3)*sin(q2))*(sin(q1)*sin(q2)*sin(q3) - cos(q2)*cos(q3)*sin(q1)) - Ixx3*(cos(q1)*cos(q2)*cos(q3) - cos(q1)*sin(q2)*sin(q3))*(cos(q2)*sin(q1)*sin(q3) + cos(q3)*sin(q1)*sin(q2)) - Iyy3*(cos(q1)*cos(q2)*sin(q3) + cos(q1)*cos(q3)*sin(q2))*(sin(q1)*sin(q2)*sin(q3) - cos(q2)*cos(q3)*sin(q1)) + Iyy3*(cos(q1)*cos(q2)*cos(q3) - cos(q1)*sin(q2)*sin(q3))*(cos(q2)*sin(q1)*sin(q3) + cos(q3)*sin(q1)*sin(q2)))))/2 - (3*sin(q1)*(cos(q1)*(Ixx3*(cos(q1)*cos(q2)*sin(q3) + cos(q1)*cos(q3)*sin(q2))*(sin(q1)*sin(q2)*sin(q3) - cos(q2)*cos(q3)*sin(q1)) - Ixx3*(cos(q1)*cos(q2)*cos(q3) - cos(q1)*sin(q2)*sin(q3))*(cos(q2)*sin(q1)*sin(q3) + cos(q3)*sin(q1)*sin(q2)) - Iyy3*(cos(q1)*cos(q2)*sin(q3) + cos(q1)*cos(q3)*sin(q2))*(sin(q1)*sin(q2)*sin(q3) - cos(q2)*cos(q3)*sin(q1)) + Iyy3*(cos(q1)*cos(q2)*cos(q3) - cos(q1)*sin(q2)*sin(q3))*(cos(q2)*sin(q1)*sin(q3) + cos(q3)*sin(q1)*sin(q2))) + sin(q1)*(2*Ixx3*(cos(q1)*cos(q2)*sin(q3) + cos(q1)*cos(q3)*sin(q2))*(cos(q1)*cos(q2)*cos(q3) - cos(q1)*sin(q2)*sin(q3)) - 2*Iyy3*(cos(q1)*cos(q2)*sin(q3) + cos(q1)*cos(q3)*sin(q2))*(cos(q1)*cos(q2)*cos(q3) - cos(q1)*sin(q2)*sin(q3)))))/2 - m3*(lc3*cos(q2)*sin(q3) + lc3*cos(q3)*sin(q2))*(cos(q2)*(l1 + l2) + lc3*cos(q2)*cos(q3) - lc3*sin(q2)*sin(q3)) + 2*m3*(lc3*cos(q1)*cos(q2)*cos(q3) - lc3*cos(q1)*sin(q2)*sin(q3))*(l2*cos(q1)*sin(q2) + lc3*cos(q1)*cos(q2)*sin(q3) + lc3*cos(q1)*cos(q3)*sin(q2)) - 2*m3*(lc3*cos(q2)*sin(q3) + lc3*cos(q3)*sin(q2))*(lc3*cos(q2)*cos(q3) - lc3*sin(q2)*sin(q3)) + 4*m3*(lc3*cos(q1)*cos(q2)*sin(q3) + lc3*cos(q1)*cos(q3)*sin(q2))*(lc3*cos(q1)*cos(q2)*cos(q3) - lc3*cos(q1)*sin(q2)*sin(q3)))];
                                                

qdd = inv(H)*(-C*qd - g_q + tau);
